simulink model "Australian14gen_forming_inertia"  (R2017b)
settings: Solver=ode23tb  StartTime=0.0  StopTime=100  FixedStep=1e-3  RelTol=1e-3  AbsTol=1e-3  EnableMultiTasking=on
PreLoadFcn:
  | dataaustralian14gen
values from neighbouring files (symbols this model uses):
  bus_v = [ 101	15 ... (first row only)    [dataaustralian14gen.m]
  c_fil = 1e-5*ones(15,1)    [dataaustralian14gen.m]
  comp = [ 1	211	0	0 ... (first row only)    [dataaustralian14gen.m]
  dist = sys.follin.dist    [main_following.m]    (also in main_forming.m = sys.formin.dist)
  Exc = [ 101	0	 200	0.1	    13.25  2.5	 0	0       0       0       0       0 ... (first row only)    [dataaustralian14gen.m]
  FH = 13    [dataaustralian14gen.m]
  FI = 1    [dataaustralian14gen.m]
  FL = .1    (= 0.1)    [dataaustralian14gen.m]
  G_data = [ 101	333.3	15	3.6	0.14	1.1	0.65	0.25	8.5     0.25	0.05	0       0       0.25	0.2 	0 ... (first row only)    [dataaustralian14gen.m]
  KH = 120    [dataaustralian14gen.m]
  KI = 10    [dataaustralian14gen.m]
  KL = 10    [dataaustralian14gen.m]
  Kvsc = 0*Kvsc    [dataaustralian14gen.m]    (also in optimgains.mat = [-4.89904313526 -21.043852985 -7.4754770322 -20.8245159401 -)
  l_fil = 5e-3*ones(15,1)    [dataaustralian14gen.m]
  line = [ 102	217	0.0084	0.0667	0.817	330	1 ... (first row only)    [dataaustralian14gen.m]
  load_mag = load_case4    [dataaustralian14gen.m]
  p = p_case4    [dataaustralian14gen.m]
  Pinit = [0.405553120017514,0.262363656270440,0.245287066765904,0.511573619715646,0.238910511748616,0.266289198874107,0.405451933295266,0.301363467877759,0.299904641553078,0.238601214125575,0.201576196829353,0.166515071179716,0.281316548159335,0.249279775700722,0.436119451429005]    [dataaustralian14gen.m]
  PSSMODEL = 1    [dataaustralian14gen.m]
  r_fil = 5e-1*ones(15,1)    [dataaustralian14gen.m]
  trans = [ 1	101	102	15	330	333.3	12	12 ... (first row only)    [dataaustralian14gen.m]
undefined symbols (not defined in the file or in its folder): D1, Delta, sys, thetavsc0
libraries: powerlib x399, Library x15, sps_avr x10, powerlib_extras x5
(part 1 of 4)
Description:
  | SimPowerSystem model of the Simplified 14-Generator model
  | of the SE Australian Power System developed by Mike Gibbard & David Vowles,
  | School of Electrical & Electronic Engineering, The university of Adelaide, south australia)
  | 
  | SimPowerSystems model and validations by Ali Moeini and Innocent Kamwa,
  | IREQ, Hydro-Québec, Canada
settings Model: Creator=IREQ  LastModifiedBy=dominic
settings DataIOCC: LimitDataPoints=on  SaveFormat=Array
settings OptimizationCC: ExpressionDepthLimit=2147483647  LifeSpan=inf
settings DebuggingCC: UnderspecifiedInitializationDetection=Classic  MergeDetectMultiDrivingBlocksExec=none  IgnoredZcDiagnostic=none  SolverPrmCheckMsg=warning  UnconnectedInputMsg=none  UnconnectedOutputMsg=none  UnconnectedLineMsg=none  StateNameClashWarn=warning  SFUnexpectedBacktrackingDiag=warning  SFNoUnconditionalDefaultTransitionDiag=warning  SFExecutionAtInitializationDiag=none
settings HardwareCC: ProdBitPerPointer=32  ProdBitPerSizeT=32  ProdBitPerPtrDiffT=32  ProdLargestAtomicFloat=None  ProdIntDivRoundTo=Undefined  ProdEndianess=Unspecified  ProdWordSize=32  ProdHWDeviceType=32-bit Generic
settings ModelReferenceCC: PropagateSignalLabelsOutOfModel=off
settings CodeAppCC: StateflowObjectComments=on
settings GRTTargetCC: TargetLangStandard=C89/C90 (ANSI)  GeneratePreprocessorConditionals=Disable all
settings ConfigComp: CovMetricSettings=dw  CovHtmlReporting=on  CovSaveCumulativeToWorkspaceVar=on  CovSaveSingleToWorkspaceVar=on  CovExternalEMLEnable=off  CovSFcnEnable=off
settings SimscapeCC: SimscapeNormalizeSystem=off

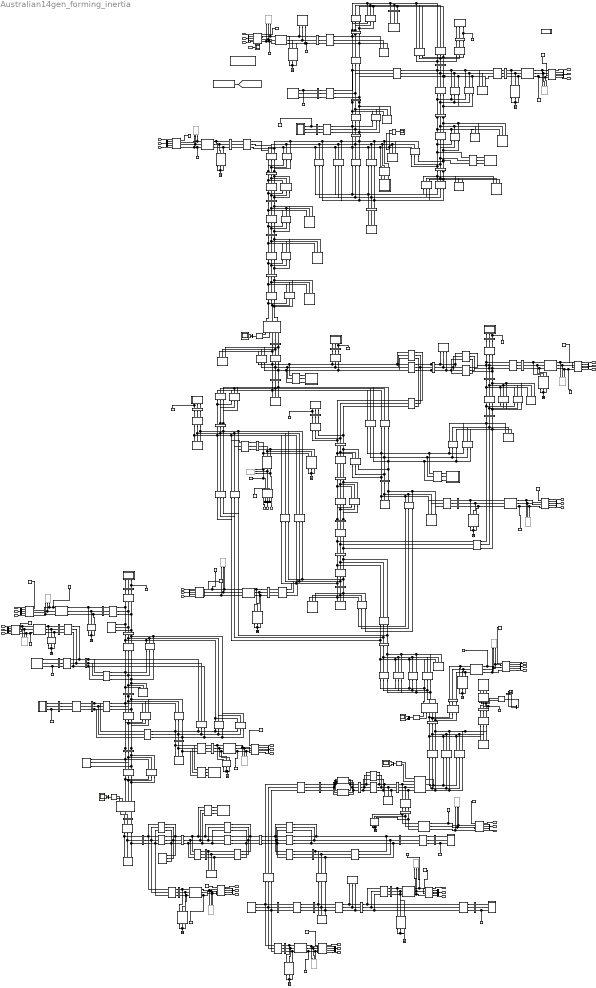
== system Australian14gen_forming_inertia ==
  1 : powerlib/Elements/Three-Phase Series RLC Branch  LConnTagsString=A|B|C  RConnTagsString=A|B|C  BranchType=C  Resistance=0  Inductance=0  Capacitance=1/(0.0337)/(2*pi*50)*(330^2/100)  Measurements=None
  15kV 1500MVA11 : powerlib/Elements/Three-Phase Series RLC Branch  LConnTagsString=A|B|C  RConnTagsString=A|B|C  BranchType=RL  Resistance=r_fil(1)  Inductance=l_fil(1)  Capacitance=[]  Measurements=None
  2 : powerlib/Elements/Three-Phase Series RLC Branch  LConnTagsString=A|B|C  RConnTagsString=A|B|C  BranchType=C  Resistance=0  Inductance=0  Capacitance=1/(0.0337)/(2*pi*50)*(330^2/100)  Measurements=None
  20kV 2000MVA : powerlib/Elements/Three-Phase Series RLC Branch  LConnTagsString=A|B|C  RConnTagsString=A|B|C  BranchType=RL  Resistance=r_fil(12)  Inductance=l_fil(12)  Capacitance=[]  Measurements=None
  20kV 2000MVA1 : powerlib/Elements/Three-Phase Series RLC Branch  LConnTagsString=A|B|C  RConnTagsString=A|B|C  BranchType=RL  Resistance=r_fil(10)  Inductance=l_fil(10)  Capacitance=[]  Measurements=None
  20kV 2000MVA10 : powerlib/Elements/Three-Phase Series RLC Branch  LConnTagsString=A|B|C  RConnTagsString=A|B|C  BranchType=RL  Resistance=r_fil(6)  Inductance=l_fil(6)  Capacitance=[]  Measurements=None
  20kV 2000MVA11 : powerlib/Elements/Three-Phase Series RLC Branch  LConnTagsString=A|B|C  RConnTagsString=A|B|C  BranchType=RL  Resistance=r_fil(14)  Inductance=l_fil(14)  Capacitance=[]  Measurements=None
  20kV 2000MVA12 : powerlib/Elements/Three-Phase Series RLC Branch  LConnTagsString=A|B|C  RConnTagsString=A|B|C  BranchType=RL  Resistance=r_fil(13)  Inductance=l_fil(13)  Capacitance=[]  Measurements=None
  20kV 2000MVA13 : powerlib/Elements/Three-Phase Series RLC Branch  LConnTagsString=A|B|C  RConnTagsString=A|B|C  BranchType=RL  Resistance=r_fil(15)  Inductance=l_fil(15)  Capacitance=[]  Measurements=None
  20kV 2000MVA14 : powerlib/Elements/Three-Phase Series RLC Branch  LConnTagsString=A|B|C  RConnTagsString=A|B|C  BranchType=C  Resistance=20^2/2000  Inductance=20^2/2000  Capacitance=c_fil(10)  Measurements=None
  20kV 2000MVA15 : powerlib/Elements/Three-Phase Series RLC Branch  LConnTagsString=A|B|C  RConnTagsString=A|B|C  BranchType=C  Resistance=20^2/2000  Inductance=20^2/2000  Capacitance=c_fil(11)  Measurements=None
  20kV 2000MVA16 : powerlib/Elements/Three-Phase Series RLC Branch  LConnTagsString=A|B|C  RConnTagsString=A|B|C  BranchType=C  Resistance=20^2/2000  Inductance=20^2/2000  Capacitance=c_fil(2)  Measurements=None
  20kV 2000MVA17 : powerlib/Elements/Three-Phase Series RLC Branch  LConnTagsString=A|B|C  RConnTagsString=A|B|C  BranchType=C  Resistance=20^2/2000  Inductance=20^2/2000  Capacitance=c_fil(3)  Measurements=None
  20kV 2000MVA18 : powerlib/Elements/Three-Phase Series RLC Branch  LConnTagsString=A|B|C  RConnTagsString=A|B|C  BranchType=C  Resistance=20^2/2000  Inductance=20^2/2000  Capacitance=c_fil(1)  Measurements=None
  20kV 2000MVA19 : powerlib/Elements/Three-Phase Series RLC Branch  LConnTagsString=A|B|C  RConnTagsString=A|B|C  BranchType=C  Resistance=20^2/2000  Inductance=20^2/2000  Capacitance=c_fil(8)  Measurements=None
  20kV 2000MVA2 : powerlib/Elements/Three-Phase Series RLC Branch  LConnTagsString=A|B|C  RConnTagsString=A|B|C  BranchType=RL  Resistance=r_fil(11)  Inductance=l_fil(11)  Capacitance=[]  Measurements=None
  20kV 2000MVA20 : powerlib/Elements/Three-Phase Series RLC Branch  LConnTagsString=A|B|C  RConnTagsString=A|B|C  BranchType=C  Resistance=20^2/2000  Inductance=20^2/2000  Capacitance=c_fil(9)  Measurements=None
  20kV 2000MVA21 : powerlib/Elements/Three-Phase Series RLC Branch  LConnTagsString=A|B|C  RConnTagsString=A|B|C  BranchType=C  Resistance=20^2/2000  Inductance=20^2/2000  Capacitance=c_fil(12)  Measurements=None
  20kV 2000MVA22 : powerlib/Elements/Three-Phase Series RLC Branch  LConnTagsString=A|B|C  RConnTagsString=A|B|C  BranchType=C  Resistance=20^2/2000  Inductance=20^2/2000  Capacitance=c_fil(5)  Measurements=None
  20kV 2000MVA23 : powerlib/Elements/Three-Phase Series RLC Branch  LConnTagsString=A|B|C  RConnTagsString=A|B|C  BranchType=C  Resistance=20^2/2000  Inductance=20^2/2000  Capacitance=c_fil(4)  Measurements=None
  20kV 2000MVA24 : powerlib/Elements/Three-Phase Series RLC Branch  LConnTagsString=A|B|C  RConnTagsString=A|B|C  BranchType=C  Resistance=20^2/2000  Inductance=20^2/2000  Capacitance=c_fil(6)  Measurements=None
  20kV 2000MVA25 : powerlib/Elements/Three-Phase Series RLC Branch  LConnTagsString=A|B|C  RConnTagsString=A|B|C  BranchType=C  Resistance=20^2/2000  Inductance=20^2/2000  Capacitance=c_fil(7)  Measurements=None
  20kV 2000MVA26 : powerlib/Elements/Three-Phase Series RLC Branch  LConnTagsString=A|B|C  RConnTagsString=A|B|C  BranchType=C  Resistance=20^2/2000  Inductance=20^2/2000  Capacitance=c_fil(15)  Measurements=None
  20kV 2000MVA27 : powerlib/Elements/Three-Phase Series RLC Branch  LConnTagsString=A|B|C  RConnTagsString=A|B|C  BranchType=C  Resistance=20^2/2000  Inductance=20^2/2000  Capacitance=c_fil(14)  Measurements=None
  20kV 2000MVA28 : powerlib/Elements/Three-Phase Series RLC Branch  LConnTagsString=A|B|C  RConnTagsString=A|B|C  BranchType=C  Resistance=20^2/2000  Inductance=20^2/2000  Capacitance=c_fil(13)  Measurements=None
  20kV 2000MVA3 : powerlib/Elements/Three-Phase Series RLC Branch  LConnTagsString=A|B|C  RConnTagsString=A|B|C  BranchType=RL  Resistance=r_fil(2)  Inductance=l_fil(2)  Capacitance=[]  Measurements=None
  20kV 2000MVA4 : powerlib/Elements/Three-Phase Series RLC Branch  LConnTagsString=A|B|C  RConnTagsString=A|B|C  BranchType=RL  Resistance=r_fil(3)  Inductance=l_fil(3)  Capacitance=[]  Measurements=None
  20kV 2000MVA5 : powerlib/Elements/Three-Phase Series RLC Branch  LConnTagsString=A|B|C  RConnTagsString=A|B|C  BranchType=RL  Resistance=r_fil(5)  Inductance=l_fil(5)  Capacitance=[]  Measurements=None
  20kV 2000MVA6 : powerlib/Elements/Three-Phase Series RLC Branch  LConnTagsString=A|B|C  RConnTagsString=A|B|C  BranchType=RL  Resistance=r_fil(4)  Inductance=l_fil(4)  Capacitance=[]  Measurements=None
  20kV 2000MVA7 : powerlib/Elements/Three-Phase Series RLC Branch  LConnTagsString=A|B|C  RConnTagsString=A|B|C  BranchType=RL  Resistance=r_fil(9)  Inductance=l_fil(9)  Capacitance=[]  Measurements=None
  20kV 2000MVA8 : powerlib/Elements/Three-Phase Series RLC Branch  LConnTagsString=A|B|C  RConnTagsString=A|B|C  BranchType=RL  Resistance=r_fil(8)  Inductance=l_fil(8)  Capacitance=[]  Measurements=None
  20kV 2000MVA9 : powerlib/Elements/Three-Phase Series RLC Branch  LConnTagsString=A|B|C  RConnTagsString=A|B|C  BranchType=RL  Resistance=r_fil(7)  Inductance=l_fil(7)  Capacitance=[]  Measurements=None
  3-Phase Active & Reactive Power (Phasor Type){1..5} (5 alike) : powerlib_extras/Phasor Library/3-Phase Active & Reactive Power (Phasor Type)
  3-Phase Dynamic Load3 : powerlib/Elements/Three-Phase Dynamic Load  NominalVoltage=[ 15e3 50 ]  ActiveReactivePowers=[-5.4e+08 -4.56e+06]  PositiveSequence=[0.999196 -2.87767]  ExternalControl=off  NpNq="[0  0]"  TimeConstants=[0 0 0 0]  MinimumVoltage=0.01  Tfilter=1e-2  LoadFlowParameters=[4 50000000 0 0 25000000]
      settings: SourceProductName=Simscape Power Systems  SourceProductBaseCode=PS
  3-Phase Dynamic Load4 : powerlib/Elements/Three-Phase Dynamic Load  NominalVoltage=[ 15e3 50 ]  ActiveReactivePowers=[-1000 -8.47033e-14]  PositiveSequence=[1.08335 6.60259]  ExternalControl=off  NpNq="[0  0]"  TimeConstants=[0 0 0 0]  MinimumVoltage=0.01  Tfilter=1e-2  LoadFlowParameters=[4 50000000 0 0 25000000]
      settings: SourceProductName=Simscape Power Systems  SourceProductBaseCode=PS
  B101 : powerlib/Measurements/Three-Phase V-I Measurement  VoltageMeasurement=phase-to-ground  SetLabelV=on  LabelV=Vabc_B101  Vpu=off  VpuLL=off  CurrentMeasurement=no  SetLabelI=on  LabelI=Iabc_B101  Ipu=off  Pbase=100e6  Vbase=bus_v(1,2)*e3  OutputType=Magnitude  PhasorSimulation=on  PSBequivalent=0
  B102 : powerlib/Measurements/Three-Phase V-I Measurement  VoltageMeasurement=phase-to-ground  SetLabelV=on  LabelV=Vabc_B102  Vpu=off  VpuLL=off  CurrentMeasurement=yes  SetLabelI=on  LabelI=Iabc_B102  Ipu=off  Pbase=100e6  Vbase=bus_v(2,2)*e3  OutputType=Complex  PhasorSimulation=on  PSBequivalent=0
  B102_vi : powerlib/Measurements/Three-Phase V-I Measurement  VoltageMeasurement=phase-to-phase  SetLabelV=on  LabelV=Vabc_B102_vi  Vpu=off  VpuLL=off  CurrentMeasurement=no  SetLabelI=on  LabelI=Iabc_B101  Ipu=off  Pbase=100e6  Vbase=bus_v(1,2)*e3  OutputType=Complex  PhasorSimulation=on  PSBequivalent=0
  B201 : powerlib/Measurements/Three-Phase V-I Measurement  VoltageMeasurement=phase-to-phase  SetLabelV=on  LabelV=Vabc_B201  Vpu=off  VpuLL=off  CurrentMeasurement=no  SetLabelI=on  LabelI=Iabc_B201  Ipu=off  Pbase=100e6  Vbase=bus_v(3,2)*e3  OutputType=Complex  PhasorSimulation=on  PSBequivalent=0
  B202 : powerlib/Measurements/Three-Phase V-I Measurement  VoltageMeasurement=phase-to-phase  SetLabelV=on  LabelV=Vabc_B202  Vpu=off  VpuLL=off  CurrentMeasurement=no  SetLabelI=on  LabelI=Iabc_B202  Ipu=off  Pbase=100e6  Vbase=bus_v(4,2)*e3  OutputType=Complex  PhasorSimulation=on  PSBequivalent=0
  B203 : powerlib/Measurements/Three-Phase V-I Measurement  VoltageMeasurement=phase-to-phase  SetLabelV=on  LabelV=Vabc_B203  Vpu=off  VpuLL=off  CurrentMeasurement=no  SetLabelI=on  LabelI=Iabc_B203  Ipu=off  Pbase=100e6  Vbase=bus_v(5,2)*e3  OutputType=Complex  PhasorSimulation=on  PSBequivalent=0
  B204 : powerlib/Measurements/Three-Phase V-I Measurement  VoltageMeasurement=phase-to-phase  SetLabelV=on  LabelV=Vabc_B204  Vpu=off  VpuLL=off  CurrentMeasurement=no  SetLabelI=on  LabelI=Iabc_B204  Ipu=off  Pbase=100e6  Vbase=bus_v(6,2)*e3  OutputType=Complex  PhasorSimulation=on  PSBequivalent=0
  B205 : powerlib/Measurements/Three-Phase V-I Measurement  VoltageMeasurement=phase-to-ground  SetLabelV=on  LabelV=Vabc_B205  Vpu=off  VpuLL=off  CurrentMeasurement=yes  SetLabelI=on  LabelI=Iabc_B205  Ipu=off  Pbase=100e6  Vbase=bus_v(7,2)*e3  OutputType=Complex  PhasorSimulation=on  PSBequivalent=0
  B206 : powerlib/Measurements/Three-Phase V-I Measurement  VoltageMeasurement=phase-to-ground  SetLabelV=on  LabelV=Vabc_B206  Vpu=off  VpuLL=off  CurrentMeasurement=yes  SetLabelI=on  LabelI=Iabc_B206  Ipu=off  Pbase=100e6  Vbase=bus_v(8,2)*e3  OutputType=Complex  PhasorSimulation=on  PSBequivalent=0
  B207 : powerlib/Measurements/Three-Phase V-I Measurement  VoltageMeasurement=phase-to-ground  SetLabelV=on  LabelV=Vabc_B207  Vpu=off  VpuLL=off  CurrentMeasurement=yes  SetLabelI=on  LabelI=Iabc_B207  Ipu=off  Pbase=100e6  Vbase=138e3  OutputType=Complex  PhasorSimulation=on  PSBequivalent=0
  B208 : powerlib/Measurements/Three-Phase V-I Measurement  VoltageMeasurement=phase-to-ground  SetLabelV=on  LabelV=Vabc_B208  Vpu=off  VpuLL=off  CurrentMeasurement=yes  SetLabelI=on  LabelI=Iabc_B208  Ipu=off  Pbase=100e6  Vbase=138e3  OutputType=Complex  PhasorSimulation=on  PSBequivalent=0
  B208_vi : powerlib/Measurements/Three-Phase V-I Measurement  VoltageMeasurement=phase-to-phase  SetLabelV=on  LabelV=Vabc_B208_vi  Vpu=off  VpuLL=off  CurrentMeasurement=no  SetLabelI=on  LabelI=Iabc_B203  Ipu=off  Pbase=100e6  Vbase=bus_v(5,2)*e3  OutputType=Complex  PhasorSimulation=on  PSBequivalent=0
  B209 : powerlib/Measurements/Three-Phase V-I Measurement  VoltageMeasurement=phase-to-ground  SetLabelV=on  LabelV=Vabc_B209  Vpu=off  VpuLL=off  CurrentMeasurement=yes  SetLabelI=on  LabelI=Iabc_B209  Ipu=off  Pbase=100e6  Vbase=138e3  OutputType=Complex  PhasorSimulation=on  PSBequivalent=0
  B210 : powerlib/Measurements/Three-Phase V-I Measurement  VoltageMeasurement=phase-to-ground  SetLabelV=on  LabelV=Vabc_B210  Vpu=off  VpuLL=off  CurrentMeasurement=yes  SetLabelI=on  LabelI=Iabc_B210  Ipu=off  Pbase=100e6  Vbase=138e3  OutputType=Complex  PhasorSimulation=on  PSBequivalent=0
  B211 : powerlib/Measurements/Three-Phase V-I Measurement  VoltageMeasurement=phase-to-ground  SetLabelV=on  LabelV=Vabc_B211  Vpu=off  VpuLL=off  CurrentMeasurement=yes  SetLabelI=on  LabelI=Iabc_B211  Ipu=off  Pbase=100e6  Vbase=138e3  OutputType=Complex  PhasorSimulation=on  PSBequivalent=0
  B212 : powerlib/Measurements/Three-Phase V-I Measurement  VoltageMeasurement=phase-to-ground  SetLabelV=on  LabelV=Vabc_B212  Vpu=off  VpuLL=off  CurrentMeasurement=yes  SetLabelI=on  LabelI=Iabc_B212  Ipu=off  Pbase=100e6  Vbase=138e3  OutputType=Complex  PhasorSimulation=on  PSBequivalent=0
  B212_vi : powerlib/Measurements/Three-Phase V-I Measurement  VoltageMeasurement=phase-to-phase  SetLabelV=on  LabelV=Vabc_B212_vi  Vpu=off  VpuLL=off  CurrentMeasurement=no  SetLabelI=on  LabelI=Iabc_B203  Ipu=off  Pbase=100e6  Vbase=bus_v(5,2)*e3  OutputType=Complex  PhasorSimulation=on  PSBequivalent=0
  B213 : powerlib/Measurements/Three-Phase V-I Measurement  VoltageMeasurement=phase-to-ground  SetLabelV=on  LabelV=Vabc_B213  Vpu=off  VpuLL=off  CurrentMeasurement=yes  SetLabelI=on  LabelI=Iabc_B213  Ipu=off  Pbase=100e6  Vbase=138e3  OutputType=Complex  PhasorSimulation=on  PSBequivalent=0
  B214 : powerlib/Measurements/Three-Phase V-I Measurement  VoltageMeasurement=phase-to-ground  SetLabelV=on  LabelV=Vabc_B214  Vpu=off  VpuLL=off  CurrentMeasurement=yes  SetLabelI=on  LabelI=Iabc_B214  Ipu=off  Pbase=100e6  Vbase=138e3  OutputType=Complex  PhasorSimulation=on  PSBequivalent=0
  B215 : powerlib/Measurements/Three-Phase V-I Measurement  VoltageMeasurement=phase-to-ground  SetLabelV=on  LabelV=Vabc_B215  Vpu=off  VpuLL=off  CurrentMeasurement=yes  SetLabelI=on  LabelI=Iabc_B215  Ipu=off  Pbase=100e6  Vbase=138e3  OutputType=Complex  PhasorSimulation=on  PSBequivalent=0
  B215_vi : powerlib/Measurements/Three-Phase V-I Measurement  VoltageMeasurement=phase-to-phase  SetLabelV=on  LabelV=Vabc_B215_vi  Vpu=off  VpuLL=off  CurrentMeasurement=no  SetLabelI=on  LabelI=Iabc_B215  Ipu=off  Pbase=100e6  Vbase=138e3  OutputType=Complex  PhasorSimulation=on  PSBequivalent=0
  B216 : powerlib/Measurements/Three-Phase V-I Measurement  VoltageMeasurement=phase-to-ground  SetLabelV=on  LabelV=Vabc_B216  Vpu=off  VpuLL=off  CurrentMeasurement=yes  SetLabelI=on  LabelI=Iabc_B216  Ipu=off  Pbase=100e6  Vbase=138e3  OutputType=Complex  PhasorSimulation=on  PSBequivalent=0
  B216_vi : powerlib/Measurements/Three-Phase V-I Measurement  VoltageMeasurement=phase-to-phase  SetLabelV=on  LabelV=Vabc_B216_vi  Vpu=off  VpuLL=off  CurrentMeasurement=no  SetLabelI=off  LabelI=Iabc_B216  Ipu=off  Pbase=100e6  Vbase=138e3  OutputType=Complex  PhasorSimulation=on  PSBequivalent=0
  B217 : powerlib/Measurements/Three-Phase V-I Measurement  VoltageMeasurement=phase-to-ground  SetLabelV=on  LabelV=Vabc_B217  Vpu=off  VpuLL=off  CurrentMeasurement=yes  SetLabelI=on  LabelI=Iabc_B217  Ipu=off  Pbase=100e6  Vbase=138e3  OutputType=Complex  PhasorSimulation=on  PSBequivalent=0
  B301 : powerlib/Measurements/Three-Phase V-I Measurement  VoltageMeasurement=phase-to-phase  SetLabelV=on  LabelV=Vabc_B301  Vpu=off  VpuLL=off  CurrentMeasurement=no  SetLabelI=on  LabelI=Iabc_B301  Ipu=off  Pbase=100e6  Vbase=138e3  OutputType=Complex  PhasorSimulation=on  PSBequivalent=0
  B302 : powerlib/Measurements/Three-Phase V-I Measurement  VoltageMeasurement=phase-to-phase  SetLabelV=on  LabelV=Vabc_B302  Vpu=off  VpuLL=off  CurrentMeasurement=no  SetLabelI=on  LabelI=Iabc_B302  Ipu=off  Pbase=100e6  Vbase=138e3  OutputType=Complex  PhasorSimulation=on  PSBequivalent=0
  B303 : powerlib/Measurements/Three-Phase V-I Measurement  VoltageMeasurement=phase-to-ground  SetLabelV=on  LabelV=Vabc_B303  Vpu=off  VpuLL=off  CurrentMeasurement=yes  SetLabelI=on  LabelI=Iabc_B303  Ipu=off  Pbase=100e6  Vbase=138e3  OutputType=Complex  PhasorSimulation=on  PSBequivalent=0
  B304 : powerlib/Measurements/Three-Phase V-I Measurement  VoltageMeasurement=phase-to-ground  SetLabelV=on  LabelV=Vabc_B304  Vpu=off  VpuLL=off  CurrentMeasurement=yes  SetLabelI=on  LabelI=Iabc_B304  Ipu=off  Pbase=100e6  Vbase=138e3  OutputType=Complex  PhasorSimulation=on  PSBequivalent=0
  B305 : powerlib/Measurements/Three-Phase V-I Measurement  VoltageMeasurement=phase-to-ground  SetLabelV=on  LabelV=Vabc_B305  Vpu=off  VpuLL=off  CurrentMeasurement=yes  SetLabelI=on  LabelI=Iabc_B305  Ipu=off  Pbase=100e6  Vbase=138e3  OutputType=Complex  PhasorSimulation=on  PSBequivalent=0
  B306 : powerlib/Measurements/Three-Phase V-I Measurement  VoltageMeasurement=phase-to-ground  SetLabelV=on  LabelV=Vabc_B306  Vpu=off  VpuLL=off  CurrentMeasurement=yes  SetLabelI=on  LabelI=Iabc_B306  Ipu=off  Pbase=100e6  Vbase=138e3  OutputType=Complex  PhasorSimulation=on  PSBequivalent=0
  B307 : powerlib/Measurements/Three-Phase V-I Measurement  VoltageMeasurement=phase-to-ground  SetLabelV=on  LabelV=Vabc_B307  Vpu=off  VpuLL=off  CurrentMeasurement=yes  SetLabelI=on  LabelI=Iabc_B307  Ipu=off  Pbase=100e6  Vbase=138e3  OutputType=Complex  PhasorSimulation=on  PSBequivalent=0
  B308 : powerlib/Measurements/Three-Phase V-I Measurement  VoltageMeasurement=phase-to-ground  SetLabelV=on  LabelV=Vabc_B308  Vpu=off  VpuLL=off  CurrentMeasurement=yes  SetLabelI=on  LabelI=Iabc_B308  Ipu=off  Pbase=100e6  Vbase=138e3  OutputType=Complex  PhasorSimulation=on  PSBequivalent=0
  B308_vi : powerlib/Measurements/Three-Phase V-I Measurement  VoltageMeasurement=phase-to-phase  SetLabelV=on  LabelV=Vabc_B308_vi  Vpu=off  VpuLL=off  CurrentMeasurement=no  SetLabelI=on  LabelI=Iabc_B301  Ipu=off  Pbase=100e6  Vbase=138e3  OutputType=Complex  PhasorSimulation=on  PSBequivalent=0
  B309 : powerlib/Measurements/Three-Phase V-I Measurement  VoltageMeasurement=phase-to-ground  SetLabelV=on  LabelV=Vabc_B309  Vpu=off  VpuLL=off  CurrentMeasurement=yes  SetLabelI=on  LabelI=Iabc_B309  Ipu=off  Pbase=100e6  Vbase=138e3  OutputType=Complex  PhasorSimulation=on  PSBequivalent=0
  B309_vi : powerlib/Measurements/Three-Phase V-I Measurement  VoltageMeasurement=phase-to-phase  SetLabelV=on  LabelV=Vabc_B309_vi  Vpu=off  VpuLL=off  CurrentMeasurement=no  SetLabelI=off  LabelI=Iabc_B309  Ipu=off  Pbase=100e6  Vbase=138e3  OutputType=Complex  PhasorSimulation=on  PSBequivalent=0
  B310 : powerlib/Measurements/Three-Phase V-I Measurement  VoltageMeasurement=phase-to-ground  SetLabelV=on  LabelV=Vabc_B310  Vpu=off  VpuLL=off  CurrentMeasurement=yes  SetLabelI=on  LabelI=Iabc_B310  Ipu=off  Pbase=100e6  Vbase=138e3  OutputType=Complex  PhasorSimulation=on  PSBequivalent=0
  B311 : powerlib/Measurements/Three-Phase V-I Measurement  VoltageMeasurement=phase-to-ground  SetLabelV=on  LabelV=Vabc_B311  Vpu=off  VpuLL=off  CurrentMeasurement=yes  SetLabelI=on  LabelI=Iabc_B311  Ipu=off  Pbase=100e6  Vbase=138e3  OutputType=Complex  PhasorSimulation=on  PSBequivalent=0
  B312 : powerlib/Measurements/Three-Phase V-I Measurement  VoltageMeasurement=phase-to-ground  SetLabelV=on  LabelV=Vabc_B312  Vpu=off  VpuLL=off  CurrentMeasurement=yes  SetLabelI=on  LabelI=Iabc_B312  Ipu=off  Pbase=100e6  Vbase=138e3  OutputType=Complex  PhasorSimulation=on  PSBequivalent=0
  B312_vi : powerlib/Measurements/Three-Phase V-I Measurement  VoltageMeasurement=phase-to-phase  SetLabelV=on  LabelV=Vabc_B312_vi  Vpu=off  VpuLL=off  CurrentMeasurement=no  SetLabelI=off  LabelI=Iabc_B312_vi  Ipu=off  Pbase=100e6  Vbase=138e3  OutputType=Complex  PhasorSimulation=on  PSBequivalent=0
  B313 : powerlib/Measurements/Three-Phase V-I Measurement  VoltageMeasurement=phase-to-ground  SetLabelV=on  LabelV=Vabc_B313  Vpu=off  VpuLL=off  CurrentMeasurement=yes  SetLabelI=on  LabelI=Iabc_B313  Ipu=off  Pbase=100e6  Vbase=138e3  OutputType=Complex  PhasorSimulation=on  PSBequivalent=0
  B314 : powerlib/Measurements/Three-Phase V-I Measurement  VoltageMeasurement=phase-to-ground  SetLabelV=on  LabelV=Vabc_B314  Vpu=off  VpuLL=off  CurrentMeasurement=yes  SetLabelI=on  LabelI=Iabc_B314  Ipu=off  Pbase=100e6  Vbase=138e3  OutputType=Complex  PhasorSimulation=on  PSBequivalent=0
  B314_vi : powerlib/Measurements/Three-Phase V-I Measurement  VoltageMeasurement=phase-to-phase  SetLabelV=on  LabelV=Vabc_B314_vi  Vpu=off  VpuLL=off  CurrentMeasurement=no  SetLabelI=off  LabelI=Iabc_B314_vi  Ipu=off  Pbase=100e6  Vbase=138e3  OutputType=Complex  PhasorSimulation=on  PSBequivalent=0
  B315 : powerlib/Measurements/Three-Phase V-I Measurement  VoltageMeasurement=phase-to-ground  SetLabelV=on  LabelV=Vabc_B315  Vpu=off  VpuLL=off  CurrentMeasurement=yes  SetLabelI=on  LabelI=Iabc_B315  Ipu=off  Pbase=100e6  Vbase=138e3  OutputType=Complex  PhasorSimulation=on  PSBequivalent=0
  B401 : powerlib/Measurements/Three-Phase V-I Measurement  VoltageMeasurement=phase-to-phase  SetLabelV=on  LabelV=Vabc_B401  Vpu=off  VpuLL=off  CurrentMeasurement=no  SetLabelI=on  LabelI=Iabc_B401  Ipu=off  Pbase=100e6  Vbase=138e3  OutputType=Complex  PhasorSimulation=on  PSBequivalent=0
  B402 : powerlib/Measurements/Three-Phase V-I Measurement  VoltageMeasurement=phase-to-ground  SetLabelV=on  LabelV=Vabc_B402  Vpu=off  VpuLL=off  CurrentMeasurement=no  SetLabelI=off  LabelI=Iabc_B402  Ipu=off  Pbase=100e6  Vbase=138e3  OutputType=Magnitude  PhasorSimulation=on  PSBequivalent=0
  B403_vi : powerlib/Measurements/Three-Phase V-I Measurement  VoltageMeasurement=phase-to-phase  SetLabelV=on  LabelV=Vabc_B403_vi  Vpu=off  VpuLL=off  CurrentMeasurement=no  SetLabelI=on  LabelI=Iabc_B403  Ipu=off  Pbase=100e6  Vbase=138e3  OutputType=Complex  PhasorSimulation=on  PSBequivalent=0
  B404 : powerlib/Measurements/Three-Phase V-I Measurement  VoltageMeasurement=phase-to-phase  SetLabelV=on  LabelV=Vabc_B404  Vpu=off  VpuLL=off  CurrentMeasurement=no  SetLabelI=on  LabelI=Iabc_B404  Ipu=off  Pbase=100e6  Vbase=138e3  OutputType=Complex  PhasorSimulation=on  PSBequivalent=0
  B405 : powerlib/Measurements/Three-Phase V-I Measurement  VoltageMeasurement=phase-to-ground  SetLabelV=on  LabelV=Vabc_B405  Vpu=off  VpuLL=off  CurrentMeasurement=yes  SetLabelI=on  LabelI=Iabc_B405  Ipu=off  Pbase=100e6  Vbase=138e3  OutputType=Complex  PhasorSimulation=on  PSBequivalent=0
  B405_vi : powerlib/Measurements/Three-Phase V-I Measurement  VoltageMeasurement=phase-to-phase  SetLabelV=on  LabelV=Vabc_B405_vi  Vpu=off  VpuLL=off  CurrentMeasurement=no  SetLabelI=on  LabelI=Iabc_B404  Ipu=off  Pbase=100e6  Vbase=138e3  OutputType=Complex  PhasorSimulation=on  PSBequivalent=0
  B406 : powerlib/Measurements/Three-Phase V-I Measurement  VoltageMeasurement=phase-to-ground  SetLabelV=on  LabelV=Vabc_B406  Vpu=off  VpuLL=off  CurrentMeasurement=yes  SetLabelI=on  LabelI=Iabc_B406  Ipu=off  Pbase=100e6  Vbase=138e3  OutputType=Complex  PhasorSimulation=on  PSBequivalent=0
  B407 : powerlib/Measurements/Three-Phase V-I Measurement  VoltageMeasurement=phase-to-ground  SetLabelV=on  LabelV=Vabc_B407  Vpu=off  VpuLL=off  CurrentMeasurement=yes  SetLabelI=on  LabelI=Iabc_B407  Ipu=off  Pbase=100e6  Vbase=138e3  OutputType=Complex  PhasorSimulation=on  PSBequivalent=0
  B408 : powerlib/Measurements/Three-Phase V-I Measurement  VoltageMeasurement=phase-to-ground  SetLabelV=on  LabelV=Vabc_B408  Vpu=off  VpuLL=off  CurrentMeasurement=yes  SetLabelI=on  LabelI=Iabc_B408  Ipu=off  Pbase=100e6  Vbase=138e3  OutputType=Complex  PhasorSimulation=on  PSBequivalent=0
  B409 : powerlib/Measurements/Three-Phase V-I Measurement  VoltageMeasurement=phase-to-ground  SetLabelV=on  LabelV=Vabc_B409  Vpu=off  VpuLL=off  CurrentMeasurement=yes  SetLabelI=on  LabelI=Iabc_B409  Ipu=off  Pbase=100e6  Vbase=138e3  OutputType=Complex  PhasorSimulation=on  PSBequivalent=0
  B410 : powerlib/Measurements/Three-Phase V-I Measurement  VoltageMeasurement=phase-to-ground  SetLabelV=on  LabelV=Vabc_B410  Vpu=off  VpuLL=off  CurrentMeasurement=no  SetLabelI=on  LabelI=Iabc_B410  Ipu=off  Pbase=100e6  Vbase=138e3  OutputType=Magnitude  PhasorSimulation=on  PSBequivalent=0
  B410_vi : powerlib/Measurements/Three-Phase V-I Measurement  VoltageMeasurement=phase-to-phase  SetLabelV=on  LabelV=Vabc_B410_vi  Vpu=off  VpuLL=off  CurrentMeasurement=no  SetLabelI=on  LabelI=Iabc_B401  Ipu=off  Pbase=100e6  Vbase=138e3  OutputType=Complex  PhasorSimulation=on  PSBequivalent=0
  B411 : powerlib/Measurements/Three-Phase V-I Measurement  VoltageMeasurement=phase-to-ground  SetLabelV=on  LabelV=Vabc_B411  Vpu=off  VpuLL=off  CurrentMeasurement=yes  SetLabelI=on  LabelI=Iabc_B411  Ipu=off  Pbase=100e6  Vbase=138e3  OutputType=Complex  PhasorSimulation=on  PSBequivalent=0
  B412 : powerlib/Measurements/Three-Phase V-I Measurement  VoltageMeasurement=phase-to-ground  SetLabelV=on  LabelV=Vabc_B412  Vpu=off  VpuLL=off  CurrentMeasurement=yes  SetLabelI=on  LabelI=Iabc_B412  Ipu=off  Pbase=100e6  Vbase=138e3  OutputType=Complex  PhasorSimulation=on  PSBequivalent=0
  B413 : powerlib/Measurements/Three-Phase V-I Measurement  VoltageMeasurement=phase-to-ground  SetLabelV=on  LabelV=Vabc_B413  Vpu=off  VpuLL=off  CurrentMeasurement=yes  SetLabelI=on  LabelI=Iabc_B413  Ipu=off  Pbase=100e6  Vbase=138e3  OutputType=Complex  PhasorSimulation=on  PSBequivalent=0
  B414 : powerlib/Measurements/Three-Phase V-I Measurement  VoltageMeasurement=phase-to-ground  SetLabelV=on  LabelV=Vabc_B414  Vpu=off  VpuLL=off  CurrentMeasurement=yes  SetLabelI=on  LabelI=Iabc_B414  Ipu=off  Pbase=100e6  Vbase=138e3  OutputType=Complex  PhasorSimulation=on  PSBequivalent=0
  B415 : powerlib/Measurements/Three-Phase V-I Measurement  VoltageMeasurement=phase-to-ground  SetLabelV=on  LabelV=Vabc_B415  Vpu=off  VpuLL=off  CurrentMeasurement=yes  SetLabelI=on  LabelI=Iabc_B415  Ipu=off  Pbase=100e6  Vbase=138e3  OutputType=Complex  PhasorSimulation=on  PSBequivalent=0
  B416 : powerlib/Measurements/Three-Phase V-I Measurement  VoltageMeasurement=phase-to-ground  SetLabelV=on  LabelV=Vabc_B416  Vpu=off  VpuLL=off  CurrentMeasurement=yes  SetLabelI=on  LabelI=Iabc_B416  Ipu=off  Pbase=100e6  Vbase=138e3  OutputType=Complex  PhasorSimulation=on  PSBequivalent=0
  B501 : powerlib/Measurements/Three-Phase V-I Measurement  VoltageMeasurement=phase-to-phase  SetLabelV=on  LabelV=Vabc_B501  Vpu=off  VpuLL=off  CurrentMeasurement=no  SetLabelI=on  LabelI=Iabc_B501  Ipu=off  Pbase=100e6  Vbase=138e3  OutputType=Complex  PhasorSimulation=on  PSBequivalent=0
  B502 : powerlib/Measurements/Three-Phase V-I Measurement  VoltageMeasurement=no  SetLabelV=on  LabelV=Vabc_B502  Vpu=off  VpuLL=off  CurrentMeasurement=no  SetLabelI=on  LabelI=Iabc_B502  Ipu=off  Pbase=100e6  Vbase=138e3  OutputType=Complex  PhasorSimulation=on  PSBequivalent=0
  B502_vi : powerlib/Measurements/Three-Phase V-I Measurement  VoltageMeasurement=phase-to-phase  SetLabelV=on  LabelV=Vabc_B502_vi  Vpu=off  VpuLL=off  CurrentMeasurement=no  SetLabelI=on  LabelI=Iabc_B502  Ipu=off  Pbase=100e6  Vbase=138e3  OutputType=Complex  PhasorSimulation=on  PSBequivalent=0
  B503 : powerlib/Measurements/Three-Phase V-I Measurement  VoltageMeasurement=phase-to-phase  SetLabelV=on  LabelV=Vabc_B503  Vpu=off  VpuLL=off  CurrentMeasurement=yes  SetLabelI=on  LabelI=Iabc_B503  Ipu=off  Pbase=100e6  Vbase=138e3  OutputType=Complex  PhasorSimulation=on  PSBequivalent=0
  B504 : powerlib/Measurements/Three-Phase V-I Measurement  VoltageMeasurement=phase-to-ground  SetLabelV=on  LabelV=Vabc_B504  Vpu=off  VpuLL=off  CurrentMeasurement=yes  SetLabelI=on  LabelI=Iabc_B504  Ipu=off  Pbase=100e6  Vbase=138e3  OutputType=Complex  PhasorSimulation=on  PSBequivalent=0
  B504_vi : powerlib/Measurements/Three-Phase V-I Measurement  VoltageMeasurement=phase-to-phase  SetLabelV=on  LabelV=Vabc_B504_vi  Vpu=off  VpuLL=off  CurrentMeasurement=no  SetLabelI=on  LabelI=Iabc_B502  Ipu=off  Pbase=100e6  Vbase=138e3  OutputType=Complex  PhasorSimulation=on  PSBequivalent=0
  B505 : powerlib/Measurements/Three-Phase V-I Measurement  VoltageMeasurement=phase-to-ground  SetLabelV=on  LabelV=Vabc_B505  Vpu=off  VpuLL=off  CurrentMeasurement=yes  SetLabelI=on  LabelI=Iabc_B505  Ipu=off  Pbase=100e6  Vbase=138e3  OutputType=Complex  PhasorSimulation=on  PSBequivalent=0
  B506 : powerlib/Measurements/Three-Phase V-I Measurement  VoltageMeasurement=phase-to-ground  SetLabelV=on  LabelV=Vabc_B506  Vpu=off  VpuLL=off  CurrentMeasurement=yes  SetLabelI=on  LabelI=Iabc_B506  Ipu=off  Pbase=100e6  Vbase=138e3  OutputType=Complex  PhasorSimulation=on  PSBequivalent=0
  B507 : powerlib/Measurements/Three-Phase V-I Measurement  VoltageMeasurement=phase-to-ground  SetLabelV=on  LabelV=Vabc_B507  Vpu=off  VpuLL=off  CurrentMeasurement=yes  SetLabelI=on  LabelI=Iabc_B507  Ipu=off  Pbase=100e6  Vbase=138e3  OutputType=Complex  PhasorSimulation=on  PSBequivalent=0
  B508 : powerlib/Measurements/Three-Phase V-I Measurement  VoltageMeasurement=phase-to-ground  SetLabelV=on  LabelV=Vabc_B508  Vpu=off  VpuLL=off  CurrentMeasurement=yes  SetLabelI=on  LabelI=Iabc_B508  Ipu=off  Pbase=100e6  Vbase=138e3  OutputType=Complex  PhasorSimulation=on  PSBequivalent=0
  B508_vi : powerlib/Measurements/Three-Phase V-I Measurement  VoltageMeasurement=phase-to-phase  SetLabelV=on  LabelV=Vabc_B508_vi  Vpu=off  VpuLL=off  CurrentMeasurement=no  SetLabelI=off  LabelI=Iabc_B503  Ipu=off  Pbase=100e6  Vbase=138e3  OutputType=Complex  PhasorSimulation=on  PSBequivalent=0
  B509 : powerlib/Measurements/Three-Phase V-I Measurement  VoltageMeasurement=phase-to-ground  SetLabelV=on  LabelV=Vabc_B3509  Vpu=off  VpuLL=off  CurrentMeasurement=yes  SetLabelI=on  LabelI=Iabc_B509  Ipu=off  Pbase=100e6  Vbase=138e3  OutputType=Complex  PhasorSimulation=on  PSBequivalent=0
  CPS402 : powerlib/Elements/Three-Phase Dynamic Load  NominalVoltage=[ 20e3 50 ]  ActiveReactivePowers=[-5.8e+08 1.015e+07]  PositiveSequence=[0.996609 23.9171]  ExternalControl=off  NpNq="[0  0]"  TimeConstants=[0 0 0 0]  MinimumVoltage=0.01  Tfilter=1e-2  LoadFlowParameters=[4 50000000 0 0 25000000]
      settings: SourceProductName=Simscape Power Systems  SourceProductBaseCode=PS
  CPS403 : powerlib/Elements/Three-Phase Dynamic Load  NominalVoltage=[ 20e3 50 ]  ActiveReactivePowers=[-9.6e+08 -3.808e+07]  PositiveSequence=[0.997203 23.5817]  ExternalControl=off  NpNq="[0  0]"  TimeConstants=[0 0 0 0]  MinimumVoltage=0.01  Tfilter=1e-2  LoadFlowParameters=[4 50000000 0 0 25000000]
      settings: SourceProductName=Simscape Power Systems  SourceProductBaseCode=PS
  Comp2-212 : powerlib/Elements/Three-Phase Parallel RLC Load  LConnTagsString=A|B|C  Configuration=Y (grounded)  NominalVoltage=(330000)*1  Vabc=[1e3 1e3 1e3]  Vabcp=[1e3 1e3 1e3]  NominalFrequency=50  UnbalancedPower=off  ActivePower=0  InductivePower=comp(2,3)*1e6  CapacitivePower=comp(2,4)*1e6  Pabc=[10e3 9e3 11e3]  QLabc=[100 90 110]  QCabc=[100 90 110]  Pabcp=[10e3 9e3 11e3]  QLabcp=[100 90 110]  QCabcp=[100 90 110]  Measurements=None  LoadType=constant Z
  Comp3-216 : powerlib/Elements/Three-Phase Parallel RLC Load  LConnTagsString=A|B|C  Configuration=Y (grounded)  NominalVoltage=(330000)*1  Vabc=[1e3 1e3 1e3]  Vabcp=[1e3 1e3 1e3]  NominalFrequency=50  UnbalancedPower=off  ActivePower=0  InductivePower=comp(3,3)*1e6  CapacitivePower=comp(3,4)*1e6  Pabc=[10e3 9e3 11e3]  QLabc=[100 90 110]  QCabc=[100 90 110]  Pabcp=[10e3 9e3 11e3]  QLabcp=[100 90 110]  QCabcp=[100 90 110]  Measurements=None  LoadType=constant Z
  Comp4-409 : powerlib/Elements/Three-Phase Parallel RLC Load  LConnTagsString=A|B|C  Configuration=Y (grounded)  NominalVoltage=(275000)*1  Vabc=[1e3 1e3 1e3]  Vabcp=[1e3 1e3 1e3]  NominalFrequency=50  UnbalancedPower=off  ActivePower=0  InductivePower=comp(4,3)*1e6  CapacitivePower=comp(4,4)*1e6  Pabc=[10e3 9e3 11e3]  QLabc=[100 90 110]  QCabc=[100 90 110]  Pabcp=[10e3 9e3 11e3]  QLabcp=[100 90 110]  QCabcp=[100 90 110]  Measurements=None  LoadType=constant Z
  Comp5-411 : powerlib/Elements/Three-Phase Parallel RLC Load  LConnTagsString=A|B|C  Configuration=Y (grounded)  NominalVoltage=(275000)*1  Vabc=[1e3 1e3 1e3]  Vabcp=[1e3 1e3 1e3]  NominalFrequency=50  UnbalancedPower=off  ActivePower=0  InductivePower=comp(5,3)*1e6  CapacitivePower=comp(5,4)*1e6  Pabc=[10e3 9e3 11e3]  QLabc=[100 90 110]  QCabc=[100 90 110]  Pabcp=[10e3 9e3 11e3]  QLabcp=[100 90 110]  QCabcp=[100 90 110]  Measurements=None  LoadType=constant Z
  Comp6-414 : powerlib/Elements/Three-Phase Parallel RLC Load  LConnTagsString=A|B|C  Configuration=Y (grounded)  NominalVoltage=(330000)*1  Vabc=[1e3 1e3 1e3]  Vabcp=[1e3 1e3 1e3]  NominalFrequency=50  UnbalancedPower=off  ActivePower=0  InductivePower=comp(6,3)*1e6  CapacitivePower=comp(6,4)*1e6  Pabc=[10e3 9e3 11e3]  QLabc=[100 90 110]  QCabc=[100 90 110]  Pabcp=[10e3 9e3 11e3]  QLabcp=[100 90 110]  QCabcp=[100 90 110]  Measurements=None  LoadType=constant Z
  Comp7-415 : powerlib/Elements/Three-Phase Parallel RLC Load  LConnTagsString=A|B|C  Configuration=Y (grounded)  NominalVoltage=(330000)*1  Vabc=[1e3 1e3 1e3]  Vabcp=[1e3 1e3 1e3]  NominalFrequency=50  UnbalancedPower=off  ActivePower=0  InductivePower=comp(7,3)*1e6  CapacitivePower=comp(7,4)*1e6  Pabc=[10e3 9e3 11e3]  QLabc=[100 90 110]  QCabc=[100 90 110]  Pabcp=[10e3 9e3 11e3]  QLabcp=[100 90 110]  QCabcp=[100 90 110]  Measurements=None  LoadType=constant Z
  Comp8-416 : powerlib/Elements/Three-Phase Parallel RLC Load  LConnTagsString=A|B|C  Configuration=Y (grounded)  NominalVoltage=(330000)*1  Vabc=[1e3 1e3 1e3]  Vabcp=[1e3 1e3 1e3]  NominalFrequency=50  UnbalancedPower=off  ActivePower=0  InductivePower=comp(8,3)*1e6  CapacitivePower=comp(8,4)*1e6  Pabc=[10e3 9e3 11e3]  QLabc=[100 90 110]  QCabc=[100 90 110]  Pabcp=[10e3 9e3 11e3]  QLabcp=[100 90 110]  QCabcp=[100 90 110]  Measurements=None  LoadType=constant Z
  Demux{,1..4} (5 alike) : Demux  Outputs=2
  Dist206 : Subsystem
  Dist212 : Subsystem
  Dist307 : Subsystem
  Dist410 : Subsystem
  Dist411 : Subsystem
  Dist508 : Subsystem
  G201_BPS : Subsystem
  G202_EPS : Subsystem
  G203_VPS : Subsystem
  G204_MPS : Subsystem
  G301_LPS : Subsystem
  G302_YPS : Subsystem
  G401_TPS : Subsystem
  G404_GPS : Subsystem
  G501_NPS : Subsystem
  G503_PPS : Subsystem
  Ground{,1..14} (15 alike) : powerlib/Elements/Ground  LConnTagsString=a
  INV102 : Library/INV  fn=50  Ub=15e3  Pref=Pinit(1)  ang=thetavsc0(1)  K2=Kvsc(1,1)  K1=Kvsc(2,1)
  INV208 : Library/INV  fn=50  Ub=20e3  Pref=Pinit(2)  ang=thetavsc0(2)  K2=Kvsc(1,2)  K1=Kvsc(2,2)
  INV212 : Library/INV  fn=50  Ub=20e3  Pref=Pinit(3)  ang=thetavsc0(3)  K2=Kvsc(1,3)  K1=Kvsc(2,3)
  INV215 : Library/INV  fn=50  Ub=20e3  Pref=Pinit(4)  ang=thetavsc0(4)  K2=Kvsc(1,4)  K1=Kvsc(2,4)
  INV216 : Library/INV  fn=50  Ub=20e3  Pref=Pinit(5)  ang=thetavsc0(5)  K2=Kvsc(1,5)  K1=Kvsc(2,5)
  INV308 : Library/INV  fn=50  Ub=20e3  Pref=Pinit(6)  ang=thetavsc0(6)  K2=Kvsc(1,6)  K1=Kvsc(2,6)
  INV309 : Library/INV  fn=50  Ub=15e3  Pref=Pinit(7)  ang=thetavsc0(7)  K2=Kvsc(1,7)  K1=Kvsc(2,7)
  INV312 : Library/INV  fn=50  Ub=20e3  Pref=Pinit(8)  ang=thetavsc0(8)  K2=Kvsc(1,8)  K1=Kvsc(2,8)
  INV314 : Library/INV  fn=50  Ub=20e3  Pref=Pinit(9)  ang=thetavsc0(9)  K2=Kvsc(1,9)  K1=Kvsc(2,9)
  INV403 : Library/INV  fn=50  Ub=20e3  Pref=Pinit(10)  ang=thetavsc0(10)  K2=Kvsc(1,10)  K1=Kvsc(2,10)
  INV405 : Library/INV  fn=50  Ub=20e3  Pref=Pinit(11)  ang=thetavsc0(11)  K2=Kvsc(1,11)  K1=Kvsc(2,11)
  INV410 : Library/INV  fn=50  Ub=20e3  Pref=Pinit(12)  ang=thetavsc0(12)  K2=Kvsc(1,12)  K1=Kvsc(2,12)
  INV502 : Library/INV  fn=50  Ub=20e3  Pref=Pinit(13)  ang=thetavsc0(13)  K2=Kvsc(1,13)  K1=Kvsc(2,13)
  INV504 : Library/INV  fn=50  Ub=20e3  Pref=Pinit(14)  ang=thetavsc0(14)  K2=Kvsc(1,14)  K1=Kvsc(2,14)
  INV508 : Library/INV  fn=50  Ub=15e3  Pref=Pinit(15)  ang=thetavsc0(15)  K2=Kvsc(1,15)  K1=Kvsc(2,15)
  L-1-1 : powerlib/Elements/Three-Phase PI Section Line  LConnTagsString=a|b|c  RConnTagsString=A|B|C  Frequency=50  Resistances="[ line(1,3)  line(1,3)*3]"  Inductances="[ line(1,4)  line(1,4)*3]"  Capacitances="[ line(1,5)  line(1,5)/3]"  Length=1
      settings: SourceProductName=Simscape Power Systems
  L-1-2 : powerlib/Elements/Three-Phase PI Section Line  LConnTagsString=a|b|c  RConnTagsString=A|B|C  Frequency=50  Resistances="[ line(1,3)  line(1,3)*3]"  Inductances="[ line(1,4)  line(1,4)*3]"  Capacitances="[ line(1,5)  line(1,5)/3]"  Length=1
      settings: SourceProductName=Simscape Power Systems
  L-10-1 : powerlib/Elements/Three-Phase PI Section Line  LConnTagsString=a|b|c  RConnTagsString=A|B|C  Frequency=50  Resistances="[ line(10,3)  line(10,3)*3]"  Inductances="[ line(10,4)  line(10,4)*3]"  Capacitances="[ line(10,5)  line(10,5)/3]"  Length=1
      settings: SourceProductName=Simscape Power Systems
  L-10-2 : powerlib/Elements/Three-Phase PI Section Line  LConnTagsString=a|b|c  RConnTagsString=A|B|C  Frequency=50  Resistances="[ line(10,3)  line(10,3)*3]"  Inductances="[ line(10,4)  line(10,4)*3]"  Capacitances="[ line(10,5)  line(10,5)/3]"  Length=1
      settings: SourceProductName=Simscape Power Systems
  L-11 : powerlib/Elements/Three-Phase PI Section Line  LConnTagsString=a|b|c  RConnTagsString=A|B|C  Frequency=50  Resistances="[ line(11,3)  line(11,3)*3]"  Inductances="[ line(11,4)  line(11,4)*3]"  Capacitances="[ line(11,5)  line(11,5)/3]"  Length=1
      settings: SourceProductName=Simscape Power Systems
  L-12-1 : powerlib/Elements/Three-Phase PI Section Line  LConnTagsString=a|b|c  RConnTagsString=A|B|C  Frequency=50  Resistances="[ line(12,3)  line(12,3)*3]"  Inductances="[ line(12,4)  line(12,4)*3]"  Capacitances="[ line(12,5)  line(12,5)/3]"  Length=1
      settings: SourceProductName=Simscape Power Systems
  L-12-2 : powerlib/Elements/Three-Phase PI Section Line  LConnTagsString=a|b|c  RConnTagsString=A|B|C  Frequency=50  Resistances="[ line(12,3)  line(12,3)*3]"  Inductances="[ line(12,4)  line(12,4)*3]"  Capacitances="[ line(12,5)  line(12,5)/3]"  Length=1
      settings: SourceProductName=Simscape Power Systems
  L-12-3 : powerlib/Elements/Three-Phase PI Section Line  LConnTagsString=a|b|c  RConnTagsString=A|B|C  Frequency=50  Resistances="[ line(12,3)  line(12,3)*3]"  Inductances="[ line(12,4)  line(12,4)*3]"  Capacitances="[ line(12,5)  line(12,5)/3]"  Length=1
      settings: SourceProductName=Simscape Power Systems
  L-13 : powerlib/Elements/Three-Phase PI Section Line  LConnTagsString=a|b|c  RConnTagsString=A|B|C  Frequency=50  Resistances="[ line(13,3)  line(13,3)*3]"  Inductances="[ line(13,4)  line(13,4)*3]"  Capacitances="[ line(13,5)  line(13,5)/3]"  Length=1
      settings: SourceProductName=Simscape Power Systems
  L-14-1 : powerlib/Elements/Three-Phase PI Section Line  LConnTagsString=a|b|c  RConnTagsString=A|B|C  Frequency=50  Resistances="[ line(14,3)  line(14,3)*3]"  Inductances="[ line(14,4)  line(14,4)*3]"  Capacitances="[ line(14,5)  line(14,5)/3]"  Length=1
      settings: SourceProductName=Simscape Power Systems
  L-14-2 : powerlib/Elements/Three-Phase PI Section Line  LConnTagsString=a|b|c  RConnTagsString=A|B|C  Frequency=50  Resistances="[ line(14,3)  line(14,3)*3]"  Inductances="[ line(14,4)  line(14,4)*3]"  Capacitances="[ line(14,5)  line(14,5)/3]"  Length=1
      settings: SourceProductName=Simscape Power Systems
  L-15-1 : powerlib/Elements/Three-Phase PI Section Line  LConnTagsString=a|b|c  RConnTagsString=A|B|C  Frequency=50  Resistances="[ line(15,3)  line(15,3)*3]"  Inductances="[ line(15,4)  line(15,4)*3]"  Capacitances="[ line(15,5)  line(15,5)/3]"  Length=1
      settings: SourceProductName=Simscape Power Systems
  L-15-2 : powerlib/Elements/Three-Phase PI Section Line  LConnTagsString=a|b|c  RConnTagsString=A|B|C  Frequency=50  Resistances="[ line(15,3)  line(15,3)*3]"  Inductances="[ line(15,4)  line(15,4)*3]"  Capacitances="[ line(15,5)  line(15,5)/3]"  Length=1
      settings: SourceProductName=Simscape Power Systems
  L-16 : powerlib/Elements/Three-Phase PI Section Line  LConnTagsString=a|b|c  RConnTagsString=A|B|C  Frequency=50  Resistances="[ line(16,3)  line(16,3)*3]"  Inductances="[ line(16,4)  line(16,4)*3]"  Capacitances="[ line(16,5)  line(16,5)/3]"  Length=1
      settings: SourceProductName=Simscape Power Systems
  L-17 : powerlib/Elements/Three-Phase PI Section Line  LConnTagsString=a|b|c  RConnTagsString=A|B|C  Frequency=50  Resistances="[ line(17,3)  line(17,3)*3]"  Inductances="[ line(17,4)  line(17,4)*3]"  Capacitances="[ line(17,5)  line(17,5)/3]"  Length=1
      settings: SourceProductName=Simscape Power Systems
  L-18 : powerlib/Elements/Three-Phase PI Section Line  LConnTagsString=a|b|c  RConnTagsString=A|B|C  Frequency=50  Resistances="[ line(18,3)  line(18,3)*3]"  Inductances="[ line(18,4)  line(18,4)*3]"  Capacitances="[ line(18,5)  line(18,5)/3]"  Length=1
      settings: SourceProductName=Simscape Power Systems
  L-19 : powerlib/Elements/Three-Phase PI Section Line  LConnTagsString=a|b|c  RConnTagsString=A|B|C  Frequency=50  Resistances="[ line(19,3)  line(19,3)*3]"  Inductances="[ line(19,4)  line(19,4)*3]"  Capacitances="[ line(19,5)  line(19,5)/3]"  Length=1
      settings: SourceProductName=Simscape Power Systems
  L-2-1 : powerlib/Elements/Three-Phase PI Section Line  LConnTagsString=a|b|c  RConnTagsString=A|B|C  Frequency=50  Resistances="[ line(2,3)  line(2,3)*3]"  Inductances="[ line(2,4)  line(2,4)*3]"  Capacitances="[ line(2,5)  line(2,5)/3]"  Length=1
      settings: SourceProductName=Simscape Power Systems
  L-2-2 : powerlib/Elements/Three-Phase PI Section Line  LConnTagsString=a|b|c  RConnTagsString=A|B|C  Frequency=50  Resistances="[ line(2,3)  line(2,3)*3]"  Inductances="[ line(2,4)  line(2,4)*3]"  Capacitances="[ line(2,5)  line(2,5)/3]"  Length=1
      settings: SourceProductName=Simscape Power Systems
  L-20-1 : powerlib/Elements/Three-Phase PI Section Line  LConnTagsString=a|b|c  RConnTagsString=A|B|C  Frequency=50  Resistances="[ line(20,3)  line(20,3)*3]"  Inductances="[ line(20,4)  line(20,4)*3]"  Capacitances="[ line(20,5)  line(20,5)/3]"  Length=1
      settings: SourceProductName=Simscape Power Systems
  L-20-2 : powerlib/Elements/Three-Phase PI Section Line  LConnTagsString=a|b|c  RConnTagsString=A|B|C  Frequency=50  Resistances="[ line(20,3)  line(20,3)*3]"  Inductances="[ line(20,4)  line(20,4)*3]"  Capacitances="[ line(20,5)  line(20,5)/3]"  Length=1
      settings: SourceProductName=Simscape Power Systems
  L-21-1 : powerlib/Elements/Three-Phase PI Section Line  LConnTagsString=a|b|c  RConnTagsString=A|B|C  Frequency=50  Resistances="[ line(21,3)  line(21,3)*3]"  Inductances="[ line(21,4)  line(21,4)*3]"  Capacitances="[ line(21,5)  line(21,5)/3]"  Length=1
      settings: SourceProductName=Simscape Power Systems
  L-21-2 : powerlib/Elements/Three-Phase PI Section Line  LConnTagsString=a|b|c  RConnTagsString=A|B|C  Frequency=50  Resistances="[ line(21,3)  line(21,3)*3]"  Inductances="[ line(21,4)  line(21,4)*3]"  Capacitances="[ line(21,5)  line(21,5)/3]"  Length=1
      settings: SourceProductName=Simscape Power Systems
  L-22 : powerlib/Elements/Three-Phase PI Section Line  LConnTagsString=a|b|c  RConnTagsString=A|B|C  Frequency=50  Resistances="[ line(22,3)  line(22,3)*3]"  Inductances="[ line(22,4)  line(22,4)*3]"  Capacitances="[ line(22,5)  line(22,5)/3]"  Length=1
      settings: SourceProductName=Simscape Power Systems
  L-23 : powerlib/Elements/Three-Phase PI Section Line  LConnTagsString=a|b|c  RConnTagsString=A|B|C  Frequency=50  Resistances="[ line(23,3)  line(23,3)*3]"  Inductances="[ line(23,4)  line(23,4)*3]"  Capacitances="[ line(23,5)  line(23,5)/3]"  Length=1
      settings: SourceProductName=Simscape Power Systems
  L-24-1 : powerlib/Elements/Three-Phase PI Section Line  LConnTagsString=a|b|c  RConnTagsString=A|B|C  Frequency=50  Resistances="[ line(24,3)  line(24,3)*3]"  Inductances="[ line(24,4)  line(24,4)*3]"  Capacitances="[ line(24,5)  line(24,5)/3]"  Length=1
      settings: SourceProductName=Simscape Power Systems
  L-24-2 : powerlib/Elements/Three-Phase PI Section Line  LConnTagsString=a|b|c  RConnTagsString=A|B|C  Frequency=50  Resistances="[ line(24,3)  line(24,3)*3]"  Inductances="[ line(24,4)  line(24,4)*3]"  Capacitances="[ line(24,5)  line(24,5)/3]"  Length=1
      settings: SourceProductName=Simscape Power Systems
  L-25 : powerlib/Elements/Three-Phase PI Section Line  LConnTagsString=a|b|c  RConnTagsString=A|B|C  Frequency=50  Resistances="[ line(25,3)  line(25,3)*3]"  Inductances="[ line(25,4)  line(25,4)*3]"  Capacitances="[ line(25,5)  line(25,5)/3]"  Length=1
      settings: SourceProductName=Simscape Power Systems
  L-26 : powerlib/Elements/Three-Phase PI Section Line  LConnTagsString=a|b|c  RConnTagsString=A|B|C  Frequency=50  Resistances="[ line(26,3)  line(26,3)*3]"  Inductances="[ line(26,4)  line(26,4)*3]"  Capacitances="[ line(26,5)  line(26,5)/3]"  Length=1
      settings: SourceProductName=Simscape Power Systems
  L-27-1 : powerlib/Elements/Three-Phase PI Section Line  LConnTagsString=a|b|c  RConnTagsString=A|B|C  Frequency=50  Resistances="[ line(27,3)  line(27,3)*3]"  Inductances="[ line(27,4)  line(27,4)*3]"  Capacitances="[ line(27,5)  line(27,5)/3]"  Length=1
      settings: SourceProductName=Simscape Power Systems
  L-27-2 : powerlib/Elements/Three-Phase PI Section Line  LConnTagsString=a|b|c  RConnTagsString=A|B|C  Frequency=50  Resistances="[ line(27,3)  line(27,3)*3]"  Inductances="[ line(27,4)  line(27,4)*3]"  Capacitances="[ line(27,5)  line(27,5)/3]"  Length=1
      settings: SourceProductName=Simscape Power Systems
  L-28 : powerlib/Elements/Three-Phase PI Section Line  LConnTagsString=a|b|c  RConnTagsString=A|B|C  Frequency=50  Resistances="[ line(28,3)  line(28,3)*3]"  Inductances="[ line(28,4)  line(28,4)*3]"  Capacitances="[ line(28,5)  line(28,5)/3]"  Length=1
      settings: SourceProductName=Simscape Power Systems
  L-29-1 : powerlib/Elements/Three-Phase PI Section Line  LConnTagsString=a|b|c  RConnTagsString=A|B|C  Frequency=50  Resistances="[ line(29,3)  line(29,3)*3]"  Inductances="[ line(29,4)  line(29,4)*3]"  Capacitances="[ line(29,5)  line(29,5)/3]"  Length=1
      settings: SourceProductName=Simscape Power Systems
  L-29-2 : powerlib/Elements/Three-Phase PI Section Line  LConnTagsString=a|b|c  RConnTagsString=A|B|C  Frequency=50  Resistances="[ line(29,3)  line(29,3)*3]"  Inductances="[ line(29,4)  line(29,4)*3]"  Capacitances="[ line(29,5)  line(29,5)/3]"  Length=1
      settings: SourceProductName=Simscape Power Systems
  L-3-1 : powerlib/Elements/Three-Phase PI Section Line  LConnTagsString=a|b|c  RConnTagsString=A|B|C  Frequency=50  Resistances="[ line(3,3)  line(3,3)*3]"  Inductances="[ line(3,4)  line(3,4)*3]"  Capacitances="[ line(3,5)  line(3,5)/3]"  Length=1
      settings: SourceProductName=Simscape Power Systems
  L-3-2 : powerlib/Elements/Three-Phase PI Section Line  LConnTagsString=a|b|c  RConnTagsString=A|B|C  Frequency=50  Resistances="[ line(3,3)  line(3,3)*3]"  Inductances="[ line(3,4)  line(3,4)*3]"  Capacitances="[ line(3,5)  line(3,5)/3]"  Length=1
      settings: SourceProductName=Simscape Power Systems
  L-30-1 : powerlib/Elements/Three-Phase PI Section Line  LConnTagsString=a|b|c  RConnTagsString=A|B|C  Frequency=50  Resistances="[ line(30,3)  line(30,3)*3]"  Inductances="[ line(30,4)  line(30,4)*3]"  Capacitances="[ line(30,5)  line(30,5)/3]"  Length=1
      settings: SourceProductName=Simscape Power Systems
  L-30-2 : powerlib/Elements/Three-Phase PI Section Line  LConnTagsString=a|b|c  RConnTagsString=A|B|C  Frequency=50  Resistances="[ line(30,3)  line(30,3)*3]"  Inductances="[ line(30,4)  line(30,4)*3]"  Capacitances="[ line(30,5)  line(30,5)/3]"  Length=1
      settings: SourceProductName=Simscape Power Systems
  L-32 : powerlib/Elements/Three-Phase PI Section Line  LConnTagsString=a|b|c  RConnTagsString=A|B|C  Frequency=50  Resistances="[ line(32,3)  line(32,3)*3]"  Inductances="[ line(32,4)  line(32,4)*3]"  Capacitances="[ line(32,5)  line(32,5)/3]"  Length=1
      settings: SourceProductName=Simscape Power Systems
  L-33 : powerlib/Elements/Three-Phase PI Section Line  LConnTagsString=a|b|c  RConnTagsString=A|B|C  Frequency=50  Resistances="[ line(33,3)  line(33,3)*3]"  Inductances="[ line(33,4)  line(33,4)*3]"  Capacitances="[ line(33,5)  line(33,5)/3]"  Length=1
      settings: SourceProductName=Simscape Power Systems
  L-34-1 : powerlib/Elements/Three-Phase PI Section Line  LConnTagsString=a|b|c  RConnTagsString=A|B|C  Frequency=50  Resistances="[ line(34,3)  line(34,3)*3]"  Inductances="[ line(34,4)  line(34,4)*3]"  Capacitances="[ line(34,5)  line(34,5)/3]"  Length=1
      settings: SourceProductName=Simscape Power Systems
  L-34-2 : powerlib/Elements/Three-Phase PI Section Line  LConnTagsString=a|b|c  RConnTagsString=A|B|C  Frequency=50  Resistances="[ line(34,3)  line(34,3)*3]"  Inductances="[ line(34,4)  line(34,4)*3]"  Capacitances="[ line(34,5)  line(34,5)/3]"  Length=1
      settings: SourceProductName=Simscape Power Systems
  L-35-1 : powerlib/Elements/Three-Phase PI Section Line  LConnTagsString=a|b|c  RConnTagsString=A|B|C  Frequency=50  Resistances="[ line(35,3)  line(35,3)*3]"  Inductances="[ line(35,4)  line(35,4)*3]"  Capacitances="[ line(35,5)  line(35,5)/3]"  Length=1
      settings: SourceProductName=Simscape Power Systems
  L-35-2 : powerlib/Elements/Three-Phase PI Section Line  LConnTagsString=a|b|c  RConnTagsString=A|B|C  Frequency=50  Resistances="[ line(35,3)  line(35,3)*3]"  Inductances="[ line(35,4)  line(35,4)*3]"  Capacitances="[ line(35,5)  line(35,5)/3]"  Length=1
      settings: SourceProductName=Simscape Power Systems
  L-36-1 : powerlib/Elements/Three-Phase PI Section Line  LConnTagsString=a|b|c  RConnTagsString=A|B|C  Frequency=50  Resistances="[ line(36,3)  line(36,3)*3]"  Inductances="[ line(36,4)  line(36,4)*3]"  Capacitances="[ line(36,5)  line(36,5)/3]"  Length=1
      settings: SourceProductName=Simscape Power Systems
  L-37-1 : powerlib/Elements/Three-Phase PI Section Line  LConnTagsString=a|b|c  RConnTagsString=A|B|C  Frequency=50  Resistances="[ line(37,3)  line(37,3)*3]"  Inductances="[ line(37,4)  line(37,4)*3]"  Capacitances="[ line(37,5)  line(37,5)/3]"  Length=1
      settings: SourceProductName=Simscape Power Systems
  L-37-2 : powerlib/Elements/Three-Phase PI Section Line  LConnTagsString=a|b|c  RConnTagsString=A|B|C  Frequency=50  Resistances="[ line(37,3)  line(37,3)*3]"  Inductances="[ line(37,4)  line(37,4)*3]"  Capacitances="[ line(37,5)  line(37,5)/3]"  Length=1
      settings: SourceProductName=Simscape Power Systems
  L-37-3 : powerlib/Elements/Three-Phase PI Section Line  LConnTagsString=a|b|c  RConnTagsString=A|B|C  Frequency=50  Resistances="[ line(37,3)  line(37,3)*3]"  Inductances="[ line(37,4)  line(37,4)*3]"  Capacitances="[ line(37,5)  line(37,5)/3]"  Length=1
      settings: SourceProductName=Simscape Power Systems
  L-38-1 : powerlib/Elements/Three-Phase PI Section Line  LConnTagsString=a|b|c  RConnTagsString=A|B|C  Frequency=50  Resistances="[ line(38,3)  line(38,3)*3]"  Inductances="[ line(38,4)  line(38,4)*3]"  Capacitances="[ line(38,5)  line(38,5)/3]"  Length=1
      settings: SourceProductName=Simscape Power Systems
  L-38-2 : powerlib/Elements/Three-Phase PI Section Line  LConnTagsString=a|b|c  RConnTagsString=A|B|C  Frequency=50  Resistances="[ line(38,3)  line(38,3)*3]"  Inductances="[ line(38,4)  line(38,4)*3]"  Capacitances="[ line(38,5)  line(38,5)/3]"  Length=1
      settings: SourceProductName=Simscape Power Systems
  L-39 : powerlib/Elements/Three-Phase PI Section Line  LConnTagsString=a|b|c  RConnTagsString=A|B|C  Frequency=50  Resistances="[ line(39,3)  line(39,3)*3]"  Inductances="[ line(39,4)  line(39,4)*3]"  Capacitances="[ line(39,5)  line(39,5)/3]"  Length=1
      settings: SourceProductName=Simscape Power Systems
  L-4 : powerlib/Elements/Three-Phase PI Section Line  LConnTagsString=a|b|c  RConnTagsString=A|B|C  Frequency=50  Resistances="[ line(4,3)  line(4,3)*3]"  Inductances="[ line(4,4)  line(4,4)*3]"  Capacitances="[ line(4,5)  line(4,5)/3]"  Length=1
      settings: SourceProductName=Simscape Power Systems
  L-40-1 : powerlib/Elements/Three-Phase PI Section Line  LConnTagsString=a|b|c  RConnTagsString=A|B|C  Frequency=50  Resistances="[ line(40,3)  line(40,3)*3]"  Inductances="[ line(40,4)  line(40,4)*3]"  Capacitances="[ line(40,5)  line(40,5)/3]"  Length=1
      settings: SourceProductName=Simscape Power Systems
  L-40-2 : powerlib/Elements/Three-Phase PI Section Line  LConnTagsString=a|b|c  RConnTagsString=A|B|C  Frequency=50  Resistances="[ line(40,3)  line(40,3)*3]"  Inductances="[ line(40,4)  line(40,4)*3]"  Capacitances="[ line(40,5)  line(40,5)/3]"  Length=1
      settings: SourceProductName=Simscape Power Systems
  L-41-1 : powerlib/Elements/Three-Phase PI Section Line  LConnTagsString=a|b|c  RConnTagsString=A|B|C  Frequency=50  Resistances="[ line(41,3)  line(41,3)*3]"  Inductances="[ line(41,4)  line(41,4)*3]"  Capacitances="[ line(41,5)  line(41,5)/3]"  Length=1
      settings: SourceProductName=Simscape Power Systems
  L-41-2 : powerlib/Elements/Three-Phase PI Section Line  LConnTagsString=a|b|c  RConnTagsString=A|B|C  Frequency=50  Resistances="[ line(41,3)  line(41,3)*3]"  Inductances="[ line(41,4)  line(41,4)*3]"  Capacitances="[ line(41,5)  line(41,5)/3]"  Length=1
      settings: SourceProductName=Simscape Power Systems
  L-42 : powerlib/Elements/Three-Phase PI Section Line  LConnTagsString=a|b|c  RConnTagsString=A|B|C  Frequency=50  Resistances="[ line(42,3)  line(42,3)*3]"  Inductances="[ line(42,4)  line(42,4)*3]"  Capacitances="[ line(42,5)  line(42,5)/3]"  Length=1
      settings: SourceProductName=Simscape Power Systems
  L-43-{1..4} (4 alike) : powerlib/Elements/Three-Phase PI Section Line  LConnTagsString=a|b|c  RConnTagsString=A|B|C  Frequency=50  Resistances="[ line(43,3)  line(43,3)*3]"  Inductances="[ line(43,4)  line(43,4)*3]"  Capacitances="[ line(43,5)  line(43,5)/3]"  Length=1
      settings: SourceProductName=Simscape Power Systems
  L-44-1 : powerlib/Elements/Three-Phase PI Section Line  LConnTagsString=a|b|c  RConnTagsString=A|B|C  Frequency=50  Resistances="[ line(44,3)  line(44,3)*3]"  Inductances="[ line(44,4)  line(44,4)*3]"  Capacitances="[ line(44,5)  line(44,5)/3]"  Length=1
      settings: SourceProductName=Simscape Power Systems
  L-44-2 : powerlib/Elements/Three-Phase PI Section Line  LConnTagsString=a|b|c  RConnTagsString=A|B|C  Frequency=50  Resistances="[ line(44,3)  line(44,3)*3]"  Inductances="[ line(44,4)  line(44,4)*3]"  Capacitances="[ line(44,5)  line(44,5)/3]"  Length=1
      settings: SourceProductName=Simscape Power Systems
  L-45-1 : powerlib/Elements/Three-Phase PI Section Line  LConnTagsString=a|b|c  RConnTagsString=A|B|C  Frequency=50  Resistances="[ line(45,3)  line(45,3)*3]"  Inductances="[ line(45,4)  line(45,4)*3]"  Capacitances="[ line(45,5)  line(45,5)/3]"  Length=1
      settings: SourceProductName=Simscape Power Systems
  L-45-2 : powerlib/Elements/Three-Phase PI Section Line  LConnTagsString=a|b|c  RConnTagsString=A|B|C  Frequency=50  Resistances="[ line(45,3)  line(45,3)*3]"  Inductances="[ line(45,4)  line(45,4)*3]"  Capacitances="[ line(45,5)  line(45,5)/3]"  Length=1
      settings: SourceProductName=Simscape Power Systems
  L-46-1 : powerlib/Elements/Three-Phase PI Section Line  LConnTagsString=a|b|c  RConnTagsString=A|B|C  Frequency=50  Resistances="[ line(46,3)  line(46,3)*3]"  Inductances="[ line(46,4)  line(46,4)*3]"  Capacitances="[ line(46,5)  line(46,5)/3]"  Length=1
      settings: SourceProductName=Simscape Power Systems
  L-46-2 : powerlib/Elements/Three-Phase PI Section Line  LConnTagsString=a|b|c  RConnTagsString=A|B|C  Frequency=50  Resistances="[ line(46,3)  line(46,3)*3]"  Inductances="[ line(46,4)  line(46,4)*3]"  Capacitances="[ line(46,5)  line(46,5)/3]"  Length=1
      settings: SourceProductName=Simscape Power Systems
  L-47-1 : powerlib/Elements/Three-Phase PI Section Line  LConnTagsString=a|b|c  RConnTagsString=A|B|C  Frequency=50  Resistances="[ line(47,3)  line(47,3)*3]"  Inductances="[ line(47,4)  line(47,4)*3]"  Capacitances="[ line(47,5)  line(47,5)/3]"  Length=1
      settings: SourceProductName=Simscape Power Systems
  L-47-2 : powerlib/Elements/Three-Phase PI Section Line  LConnTagsString=a|b|c  RConnTagsString=A|B|C  Frequency=50  Resistances="[ line(47,3)  line(47,3)*3]"  Inductances="[ line(47,4)  line(47,4)*3]"  Capacitances="[ line(47,5)  line(47,5)/3]"  Length=1
      settings: SourceProductName=Simscape Power Systems
  L-48-1 : powerlib/Elements/Three-Phase PI Section Line  LConnTagsString=a|b|c  RConnTagsString=A|B|C  Frequency=50  Resistances="[ line(48,3)  line(48,3)*3]"  Inductances="[ line(48,4)  line(48,4)*3]"  Capacitances="[ line(48,5)  line(48,5)/3]"  Length=1
      settings: SourceProductName=Simscape Power Systems
  L-48-2 : powerlib/Elements/Three-Phase PI Section Line  LConnTagsString=a|b|c  RConnTagsString=A|B|C  Frequency=50  Resistances="[ line(48,3)  line(48,3)*3]"  Inductances="[ line(48,4)  line(48,4)*3]"  Capacitances="[ line(48,5)  line(48,5)/3]"  Length=1
      settings: SourceProductName=Simscape Power Systems
  L-49-1 : powerlib/Elements/Three-Phase PI Section Line  LConnTagsString=a|b|c  RConnTagsString=A|B|C  Frequency=50  Resistances="[ line(49,3)  line(49,3)*3]"  Inductances="[ line(49,4)  line(49,4)*3]"  Capacitances="[ line(49,5)  line(49,5)/3]"  Length=1
      settings: SourceProductName=Simscape Power Systems
  L-49-2 : powerlib/Elements/Three-Phase PI Section Line  LConnTagsString=a|b|c  RConnTagsString=A|B|C  Frequency=50  Resistances="[ line(49,3)  line(49,3)*3]"  Inductances="[ line(49,4)  line(49,4)*3]"  Capacitances="[ line(49,5)  line(49,5)/3]"  Length=1
      settings: SourceProductName=Simscape Power Systems
  L-5-1 : powerlib/Elements/Three-Phase PI Section Line  LConnTagsString=a|b|c  RConnTagsString=A|B|C  Frequency=50  Resistances="[ line(5,3)  line(5,3)*3]"  Inductances="[ line(5,4)  line(5,4)*3]"  Capacitances="[ line(5,5)  line(5,5)/3]"  Length=1
      settings: SourceProductName=Simscape Power Systems
  L-5-2 : powerlib/Elements/Three-Phase PI Section Line  LConnTagsString=a|b|c  RConnTagsString=A|B|C  Frequency=50  Resistances="[ line(5,3)  line(5,3)*3]"  Inductances="[ line(5,4)  line(5,4)*3]"  Capacitances="[ line(5,5)  line(5,5)/3]"  Length=1
      settings: SourceProductName=Simscape Power Systems
  L-50-1 : powerlib/Elements/Three-Phase PI Section Line  LConnTagsString=a|b|c  RConnTagsString=A|B|C  Frequency=50  Resistances="[ line(50,3)  line(50,3)*3]"  Inductances="[ line(50,4)  line(50,4)*3]"  Capacitances="[ line(50,5)  line(50,5)/3]"  Length=1
      settings: SourceProductName=Simscape Power Systems
  L-51 : powerlib/Elements/Three-Phase PI Section Line  LConnTagsString=a|b|c  RConnTagsString=A|B|C  Frequency=50  Resistances="[ line(51,3)  line(51,3)*3]"  Inductances="[ line(51,4)  line(51,4)*3]"  Capacitances="[ line(51,5)  line(51,5)/3]"  Length=1
      settings: SourceProductName=Simscape Power Systems
  L-52 : powerlib/Elements/Three-Phase PI Section Line  LConnTagsString=a|b|c  RConnTagsString=A|B|C  Frequency=50  Resistances="[ line(52,3)  line(52,3)*3]"  Inductances="[ line(52,4)  line(52,4)*3]"  Capacitances="[ line(52,5)  line(52,5)/3]"  Length=1
      settings: SourceProductName=Simscape Power Systems
  L-53 : powerlib/Elements/Three-Phase PI Section Line  LConnTagsString=a|b|c  RConnTagsString=A|B|C  Frequency=50  Resistances="[ line(53,3)  line(53,3)*3]"  Inductances="[ line(53,4)  line(53,4)*3]"  Capacitances="[ line(53,5)  line(53,5)/3]"  Length=1
      settings: SourceProductName=Simscape Power Systems
  L-54 : powerlib/Elements/Three-Phase PI Section Line  LConnTagsString=a|b|c  RConnTagsString=A|B|C  Frequency=50  Resistances=[ line(54,3) line(54,3)*3]  Inductances=[ line(54,4) line(54,4)*3]  Capacitances=[ line(54,5) line(54,5)/3]  Length=1
      settings: SourceProductName=Simscape Power Systems
  L-55-1 : powerlib/Elements/Three-Phase PI Section Line  LConnTagsString=a|b|c  RConnTagsString=A|B|C  Frequency=50  Resistances=[ line(55,3) line(55,3)*3]  Inductances="[ line(55,4)  line(55,4)*3]"  Capacitances="[line(55,5)  line(55,5)/3]"  Length=1
      settings: SourceProductName=Simscape Power Systems
  L-55-2 : powerlib/Elements/Three-Phase PI Section Line  LConnTagsString=a|b|c  RConnTagsString=A|B|C  Frequency=50  Resistances=[ line(55,3) line(55,3)*3]  Inductances="[ line(55,4)  line(55,4)*3]"  Capacitances="[line(55,5)  line(55,5)/3]"  Length=1
      settings: SourceProductName=Simscape Power Systems
  L-6-1 : powerlib/Elements/Three-Phase PI Section Line  LConnTagsString=a|b|c  RConnTagsString=A|B|C  Frequency=50  Resistances="[ line(6,3)  line(6,3)*3]"  Inductances="[ line(6,4)  line(6,4)*3]"  Capacitances="[ line(6,5)  line(6,5)/3]"  Length=1
      settings: SourceProductName=Simscape Power Systems
  L-6-2 : powerlib/Elements/Three-Phase PI Section Line  LConnTagsString=a|b|c  RConnTagsString=A|B|C  Frequency=50  Resistances="[ line(6,3)  line(6,3)*3]"  Inductances="[ line(6,4)  line(6,4)*3]"  Capacitances="[ line(6,5)  line(6,5)/3]"  Length=1
      settings: SourceProductName=Simscape Power Systems
  L-7-1 : powerlib/Elements/Three-Phase PI Section Line  LConnTagsString=a|b|c  RConnTagsString=A|B|C  Frequency=50  Resistances="[ line(7,3)  line(7,3)*3]"  Inductances="[ line(7,4)  line(7,4)*3]"  Capacitances="[ line(7,5)  line(7,5)/3]"  Length=1
      settings: SourceProductName=Simscape Power Systems
  L-7-2 : powerlib/Elements/Three-Phase PI Section Line  LConnTagsString=a|b|c  RConnTagsString=A|B|C  Frequency=50  Resistances="[ line(7,3)  line(7,3)*3]"  Inductances="[ line(7,4)  line(7,4)*3]"  Capacitances="[ line(7,5)  line(7,5)/3]"  Length=1
      settings: SourceProductName=Simscape Power Systems
  L-8-1 : powerlib/Elements/Three-Phase PI Section Line  LConnTagsString=a|b|c  RConnTagsString=A|B|C  Frequency=50  Resistances="[ line(8,3)  line(8,3)*3]"  Inductances="[ line(8,4)  line(8,4)*3]"  Capacitances="[ line(8,5)  line(8,5)/3]"  Length=1
      settings: SourceProductName=Simscape Power Systems
  L-8-2 : powerlib/Elements/Three-Phase PI Section Line  LConnTagsString=a|b|c  RConnTagsString=A|B|C  Frequency=50  Resistances="[ line(8,3)  line(8,3)*3]"  Inductances="[ line(8,4)  line(8,4)*3]"  Capacitances="[ line(8,5)  line(8,5)/3]"  Length=1
      settings: SourceProductName=Simscape Power Systems
  L-9-1 : powerlib/Elements/Three-Phase PI Section Line  LConnTagsString=a|b|c  RConnTagsString=A|B|C  Frequency=50  Resistances="[ line(9,3)  line(9,3)*3]"  Inductances="[ line(9,4)  line(9,4)*3]"  Capacitances="[ line(9,5)  line(9,5)/3]"  Length=1
      settings: SourceProductName=Simscape Power Systems
  L-9-2 : powerlib/Elements/Three-Phase PI Section Line  LConnTagsString=a|b|c  RConnTagsString=A|B|C  Frequency=50  Resistances="[ line(9,3)  line(9,3)*3]"  Inductances="[ line(9,4)  line(9,4)*3]"  Capacitances="[ line(9,5)  line(9,5)/3]"  Length=1
      settings: SourceProductName=Simscape Power Systems
  Load Flow Bus1 : powerlib/Measurements/Load Flow Bus  LConnTagsString=a  Phases=single  Connectors=on one side  ID=B403_vsw  Vbase=20e3  Vref=1  Vangle=0  VLF=0.9972  VLFb=1  VLFc=1  angleLF=23.58  angleLFb=0  angleLFc=0
      settings: AttributesFormatString=%<ID>\n%<Vbase>V\n%<VLF>pu\n%<angleLF>deg.  SourceProductName=Simscape Power Systems
  Load Flow Bus10 : powerlib/Measurements/Load Flow Bus  LConnTagsString=a  Phases=single  Connectors=on one side  ID=B301  Vbase=20e3  Vref=1  Vangle=0  VLF=1  VLFb=1  VLFc=1  angleLF=-10.04  angleLFb=0  angleLFc=0
      settings: AttributesFormatString=%<ID>\n%<Vbase>V\n%<VLF>pu\n%<angleLF>deg.  SourceProductName=Simscape Power Systems
  Load Flow Bus11 : powerlib/Measurements/Load Flow Bus  LConnTagsString=a  Phases=single  Connectors=on one side  ID=B302  Vbase=20e3  Vref=1  Vangle=0  VLF=1  VLFb=1  VLFc=1  angleLF=-18.96  angleLFb=0  angleLFc=0
      settings: AttributesFormatString=%<ID>\n%<Vbase>V\n%<VLF>pu\n%<angleLF>deg.  SourceProductName=Simscape Power Systems
  Load Flow Bus12 : powerlib/Measurements/Load Flow Bus  LConnTagsString=a  Phases=single  Connectors=on one side  ID=B503  Vbase=15e3  Vref=1  Vangle=0  VLF=1  VLFb=1  VLFc=1  angleLF=-38.47  angleLFb=0  angleLFc=0
      settings: AttributesFormatString=%<ID>\n%<Vbase>V\n%<VLF>pu\n%<angleLF>deg.  SourceProductName=Simscape Power Systems
  Load Flow Bus13 : powerlib/Measurements/Load Flow Bus  LConnTagsString=a  Phases=single  Connectors=on one side  ID=B502  Vbase=15e3  Vref=1  Vangle=0  VLF=0.9992  VLFb=1  VLFc=1  angleLF=-2.878  angleLFb=0  angleLFc=0
      settings: AttributesFormatString=%<ID>\n%<Vbase>V\n%<VLF>pu\n%<angleLF>deg.  SourceProductName=Simscape Power Systems
  Load Flow Bus14 : powerlib/Measurements/Load Flow Bus  LConnTagsString=a  Phases=single  Connectors=on one side  ID=B501  Vbase=20e3  Vref=1  Vangle=0  VLF=1  VLFb=1  VLFc=1  angleLF=-34.56  angleLFb=0  angleLFc=0
      settings: AttributesFormatString=%<ID>\n%<Vbase>V\n%<VLF>pu\n%<angleLF>deg.  SourceProductName=Simscape Power Systems
  Load Flow Bus15 : powerlib/Measurements/Load Flow Bus  LConnTagsString=a  Phases=single  Connectors=on one side  ID=B403  Vbase=20e3  Vref=1  Vangle=0  VLF=0.9972  VLFb=1  VLFc=1  angleLF=23.58  angleLFb=0  angleLFc=0
      settings: AttributesFormatString=%<ID>\n%<Vbase>V\n%<VLF>pu\n%<angleLF>deg.  SourceProductName=Simscape Power Systems
  Load Flow Bus16 : powerlib/Measurements/Load Flow Bus  LConnTagsString=a  Phases=single  Connectors=on one side  ID=B410_vsw  Vbase=20e3  Vref=1  Vangle=0  VLF=1  VLFb=1  VLFc=1  angleLF=2.825  angleLFb=0  angleLFc=0
      settings: AttributesFormatString=%<ID>\n%<Vbase>V\n%<VLF>pu\n%<angleLF>deg.  SourceProductName=Simscape Power Systems
  Load Flow Bus17 : powerlib/Measurements/Load Flow Bus  LConnTagsString=a  Phases=single  Connectors=on one side  ID=B504_vsw  Vbase=20e3  Vref=1  Vangle=0  VLF=1  VLFb=1  VLFc=1  angleLF=-12.45  angleLFb=0  angleLFc=0
      settings: AttributesFormatString=%<ID>\n%<Vbase>V\n%<VLF>pu\n%<angleLF>deg.  SourceProductName=Simscape Power Systems
  Load Flow Bus18 : powerlib/Measurements/Load Flow Bus  LConnTagsString=a  Phases=single  Connectors=on one side  ID=B502_vsw  Vbase=20e3  Vref=1  Vangle=0  VLF=1  VLFb=1  VLFc=1  angleLF=-12.71  angleLFb=0  angleLFc=0
      settings: AttributesFormatString=%<ID>\n%<Vbase>V\n%<VLF>pu\n%<angleLF>deg.  SourceProductName=Simscape Power Systems
  Load Flow Bus19 : powerlib/Measurements/Load Flow Bus  LConnTagsString=a  Phases=single  Connectors=on one side  ID=B508_vsw  Vbase=15e3  Vref=1  Vangle=0  VLF=1  VLFb=1  VLFc=1  angleLF=-14.76  angleLFb=0  angleLFc=0
      settings: AttributesFormatString=%<ID>\n%<Vbase>V\n%<VLF>pu\n%<angleLF>deg.  SourceProductName=Simscape Power Systems
  Load Flow Bus2 : powerlib/Measurements/Load Flow Bus  LConnTagsString=a  Phases=single  Connectors=on one side  ID=B404  Vbase=20e3  Vref=1  Vangle=0  VLF=1  VLFb=1  VLFc=1  angleLF=-13.1  angleLFb=0  angleLFc=0
      settings: AttributesFormatString=%<ID>\n%<Vbase>V\n%<VLF>pu\n%<angleLF>deg.  SourceProductName=Simscape Power Systems
  Load Flow Bus20 : powerlib/Measurements/Load Flow Bus  LConnTagsString=a  Phases=single  Connectors=on one side  ID=B308_vsw  Vbase=20e3  Vref=1  Vangle=0  VLF=1  VLFb=1  VLFc=1  angleLF=-6.338  angleLFb=0  angleLFc=0
      settings: AttributesFormatString=%<ID>\n%<Vbase>V\n%<VLF>pu\n%<angleLF>deg.  SourceProductName=Simscape Power Systems
  Load Flow Bus21 : powerlib/Measurements/Load Flow Bus  LConnTagsString=a  Phases=single  Connectors=on one side  ID=B314_vsw  Vbase=20e3  Vref=1  Vangle=0  VLF=1  VLFb=1  VLFc=1  angleLF=-1.099  angleLFb=0  angleLFc=0
      settings: AttributesFormatString=%<ID>\n%<Vbase>V\n%<VLF>pu\n%<angleLF>deg.  SourceProductName=Simscape Power Systems
  Load Flow Bus22 : powerlib/Measurements/Load Flow Bus  LConnTagsString=a  Phases=single  Connectors=on one side  ID=B312_vsw  Vbase=20e3  Vref=1  Vangle=0  VLF=1  VLFb=1  VLFc=1  angleLF=3.684  angleLFb=0  angleLFc=0
      settings: AttributesFormatString=%<ID>\n%<Vbase>V\n%<VLF>pu\n%<angleLF>deg.  SourceProductName=Simscape Power Systems
  Load Flow Bus23 : powerlib/Measurements/Load Flow Bus  LConnTagsString=a  Phases=single  Connectors=on one side  ID=B309_vsw  Vbase=15e3  Vref=1  Vangle=0  VLF=1  VLFb=1  VLFc=1  angleLF=4.793  angleLFb=0  angleLFc=0
      settings: AttributesFormatString=%<ID>\n%<Vbase>V\n%<VLF>pu\n%<angleLF>deg.  SourceProductName=Simscape Power Systems
  Load Flow Bus24 : powerlib/Measurements/Load Flow Bus  LConnTagsString=a  Phases=single  Connectors=on one side  ID=B102_vsw  Vbase=15e3  Vref=1  Vangle=0  VLF=1  VLFb=1  VLFc=1  angleLF=6.617  angleLFb=0  angleLFc=0
      settings: AttributesFormatString=%<ID>\n%<Vbase>V\n%<VLF>pu\n%<angleLF>deg.  SourceProductName=Simscape Power Systems
  Load Flow Bus25 : powerlib/Measurements/Load Flow Bus  LConnTagsString=a  Phases=single  Connectors=on one side  ID=B216_vsw  Vbase=20e3  Vref=1  Vangle=0  VLF=1  VLFb=1  VLFc=1  angleLF=14.02  angleLFb=0  angleLFc=0
      settings: AttributesFormatString=%<ID>\n%<Vbase>V\n%<VLF>pu\n%<angleLF>deg.  SourceProductName=Simscape Power Systems
  Load Flow Bus26 : powerlib/Measurements/Load Flow Bus  LConnTagsString=a  Phases=single  Connectors=on one side  ID=B215_vsw  Vbase=20e3  Vref=1  Vangle=0  VLF=1  VLFb=1  VLFc=1  angleLF=23.87  angleLFb=0  angleLFc=0
      settings: AttributesFormatString=%<ID>\n%<Vbase>V\n%<VLF>pu\n%<angleLF>deg.  SourceProductName=Simscape Power Systems
  Load Flow Bus27 : powerlib/Measurements/Load Flow Bus  LConnTagsString=a  Phases=single  Connectors=on one side  ID=B212_vsw  Vbase=20e3  Vref=1  Vangle=0  VLF=1  VLFb=1  VLFc=1  angleLF=15.52  angleLFb=0  angleLFc=0
      settings: AttributesFormatString=%<ID>\n%<Vbase>V\n%<VLF>pu\n%<angleLF>deg.  SourceProductName=Simscape Power Systems
  Load Flow Bus28 : powerlib/Measurements/Load Flow Bus  LConnTagsString=a  Phases=single  Connectors=on one side  ID=B208_vsw  Vbase=20e3  Vref=1  Vangle=0  VLF=1  VLFb=1  VLFc=1  angleLF=21.27  angleLFb=0  angleLFc=0
      settings: AttributesFormatString=%<ID>\n%<Vbase>V\n%<VLF>pu\n%<angleLF>deg.  SourceProductName=Simscape Power Systems
  Load Flow Bus29 : powerlib/Measurements/Load Flow Bus  LConnTagsString=a  Phases=single  Connectors=on one side  ID=B405_vsw  Vbase=20e3  Vref=1  Vangle=0  VLF=0.9972  VLFb=1  VLFc=1  angleLF=23.58  angleLFb=0  angleLFc=0
      settings: AttributesFormatString=%<ID>\n%<Vbase>V\n%<VLF>pu\n%<angleLF>deg.  SourceProductName=Simscape Power Systems
  Load Flow Bus3 : powerlib/Measurements/Load Flow Bus  LConnTagsString=a  Phases=single  Connectors=on one side  ID=B402  Vbase=20e3  Vref=1  Vangle=0  VLF=0.9966  VLFb=1  VLFc=1  angleLF=23.92  angleLFb=0  angleLFc=0
      settings: AttributesFormatString=%<ID>\n%<Vbase>V\n%<VLF>pu\n%<angleLF>deg.  SourceProductName=Simscape Power Systems
  Load Flow Bus4 : powerlib/Measurements/Load Flow Bus  LConnTagsString=a  Phases=single  Connectors=on one side  ID=B401  Vbase=20e3  Vref=1  Vangle=0  VLF=1  VLFb=1  VLFc=1  angleLF=-21.06  angleLFb=0  angleLFc=0
      settings: AttributesFormatString=%<ID>\n%<Vbase>V\n%<VLF>pu\n%<angleLF>deg.  SourceProductName=Simscape Power Systems
  Load Flow Bus5 : powerlib/Measurements/Load Flow Bus  LConnTagsString=a  Phases=single  Connectors=on one side  ID=B203  Vbase=20e3  Vref=1  Vangle=0  VLF=1  VLFb=1  VLFc=1  angleLF=-0.543  angleLFb=0  angleLFc=0
      settings: AttributesFormatString=%<ID>\n%<Vbase>V\n%<VLF>pu\n%<angleLF>deg.  SourceProductName=Simscape Power Systems
  Load Flow Bus6 : powerlib/Measurements/Load Flow Bus  LConnTagsString=a  Phases=single  Connectors=on one side  ID=B201  Vbase=20e3  Vref=1  Vangle=0  VLF=1  VLFb=1  VLFc=1  angleLF=3.923  angleLFb=0  angleLFc=0
      settings: AttributesFormatString=%<ID>\n%<Vbase>V\n%<VLF>pu\n%<angleLF>deg.  SourceProductName=Simscape Power Systems
  Load Flow Bus7 : powerlib/Measurements/Load Flow Bus  LConnTagsString=a  Phases=single  Connectors=on one side  ID=B202  Vbase=20e3  Vref=1  Vangle=0  VLF=1  VLFb=1  VLFc=1  angleLF=-0.2053  angleLFb=0  angleLFc=0
      settings: AttributesFormatString=%<ID>\n%<Vbase>V\n%<VLF>pu\n%<angleLF>deg.  SourceProductName=Simscape Power Systems
  Load Flow Bus8 : powerlib/Measurements/Load Flow Bus  LConnTagsString=a  Phases=single  Connectors=on one side  ID=B204  Vbase=20e3  Vref=1  Vangle=0  VLF=1  VLFb=1  VLFc=1  angleLF=0  angleLFb=0  angleLFc=0
      settings: AttributesFormatString=%<ID>\n%<Vbase>V\n%<VLF>pu\n%<angleLF>deg.  SourceProductName=Simscape Power Systems
  Load Flow Bus9 : powerlib/Measurements/Load Flow Bus  LConnTagsString=a  Phases=single  Connectors=on one side  ID=B101  Vbase=15e3  Vref=1  Vangle=0  VLF=1.083  VLFb=1  VLFc=1  angleLF=6.603  angleLFb=0  angleLFc=0
      settings: AttributesFormatString=%<ID>\n%<Vbase>V\n%<VLF>pu\n%<angleLF>deg.  SourceProductName=Simscape Power Systems
  Load1 : powerlib/Elements/Three-Phase Parallel RLC Load  LConnTagsString=A|B|C  Configuration=Y (grounded)  NominalVoltage=(356540)*1.00295  Vabc=[1e3 1e3 1e3]  Vabcp=[1e3 1e3 1e3]  NominalFrequency=50  UnbalancedPower=off  ActivePower=load_mag(1,2)*1e6  InductivePower=load_mag(1,3)*1e6  CapacitivePower=0  Pabc=[10e3 9e3 11e3]  QLabc=[100 90 110]  QCabc=[100 90 110]  Pabcp=[10e3 9e3 11e3]  QLabcp=[100 90 110]  QCabcp=[100 90 110]  Measurements=None  LoadType=constant PQ
  Load10 : powerlib/Elements/Three-Phase Parallel RLC Load  LConnTagsString=A|B|C  Configuration=Y (grounded)  NominalVoltage=(346286)*1.00201  Vabc=[1e3 1e3 1e3]  Vabcp=[1e3 1e3 1e3]  NominalFrequency=50  UnbalancedPower=off  ActivePower=load_mag(10,2)*1e6  InductivePower=load_mag(10,3)*1e6  CapacitivePower=0  Pabc=[10e3 9e3 11e3]  QLabc=[100 90 110]  QCabc=[100 90 110]  Pabcp=[10e3 9e3 11e3]  QLabcp=[100 90 110]  QCabcp=[100 90 110]  Measurements=None  LoadType=constant PQ
  Load11 : powerlib/Elements/Three-Phase Parallel RLC Load  LConnTagsString=A|B|C  Configuration=Y (grounded)  NominalVoltage=(511149)*1.0019  Vabc=[1e3 1e3 1e3]  Vabcp=[1e3 1e3 1e3]  NominalFrequency=50  UnbalancedPower=off  ActivePower=load_mag(11,2)*1e6  InductivePower=load_mag(11,3)*1e6  CapacitivePower=0  Pabc=[10e3 9e3 11e3]  QLabc=[100 90 110]  QCabc=[100 90 110]  Pabcp=[10e3 9e3 11e3]  QLabcp=[100 90 110]  QCabcp=[100 90 110]  Measurements=None  LoadType=constant PQ
  Load12 : powerlib/Elements/Three-Phase Parallel RLC Load  LConnTagsString=A|B|C  Configuration=Y (grounded)  NominalVoltage=(512503)*1.00192  Vabc=[1e3 1e3 1e3]  Vabcp=[1e3 1e3 1e3]  NominalFrequency=50  UnbalancedPower=off  ActivePower=load_mag(12,2)*1e6  InductivePower=load_mag(12,3)*1e6  CapacitivePower=0  Pabc=[10e3 9e3 11e3]  QLabc=[100 90 110]  QCabc=[100 90 110]  Pabcp=[10e3 9e3 11e3]  QLabcp=[100 90 110]  QCabcp=[100 90 110]  Measurements=None  LoadType=constant PQ
  Load13 : powerlib/Elements/Three-Phase Parallel RLC Load  LConnTagsString=A|B|C  Configuration=Y (grounded)  NominalVoltage=(529566)*1.00301  Vabc=[1e3 1e3 1e3]  Vabcp=[1e3 1e3 1e3]  NominalFrequency=50  UnbalancedPower=off  ActivePower=load_mag(13,2)*1e6  InductivePower=load_mag(13,3)*1e6  CapacitivePower=0  Pabc=[10e3 9e3 11e3]  QLabc=[100 90 110]  QCabc=[100 90 110]  Pabcp=[10e3 9e3 11e3]  QLabcp=[100 90 110]  QCabcp=[100 90 110]  Measurements=None  LoadType=constant PQ
  Load14 : powerlib/Elements/Three-Phase Parallel RLC Load  LConnTagsString=A|B|C  Configuration=Y (grounded)  NominalVoltage=(357825)*1.00308  Vabc=[1e3 1e3 1e3]  Vabcp=[1e3 1e3 1e3]  NominalFrequency=50  UnbalancedPower=off  ActivePower=load_mag(14,2)*1e6  InductivePower=load_mag(14,3)*1e6  CapacitivePower=0  Pabc=[10e3 9e3 11e3]  QLabc=[100 90 110]  QCabc=[100 90 110]  Pabcp=[10e3 9e3 11e3]  QLabcp=[100 90 110]  QCabcp=[100 90 110]  Measurements=None  LoadType=constant PQ
  Load15 : powerlib/Elements/Three-Phase Parallel RLC Load  LConnTagsString=A|B|C  Configuration=Y (grounded)  NominalVoltage=(220026)*1.00158  Vabc=[1e3 1e3 1e3]  Vabcp=[1e3 1e3 1e3]  NominalFrequency=50  UnbalancedPower=off  ActivePower=load_mag(15,2)*1e6  InductivePower=load_mag(15,3)*1e6  CapacitivePower=0  Pabc=[10e3 9e3 11e3]  QLabc=[100 90 110]  QCabc=[100 90 110]  Pabcp=[10e3 9e3 11e3]  QLabcp=[100 90 110]  QCabcp=[100 90 110]  Measurements=None  LoadType=constant PQ
  Load16 : powerlib/Elements/Three-Phase Parallel RLC Load  LConnTagsString=A|B|C  Configuration=Y (grounded)  NominalVoltage=(218962)*1.00201  Vabc=[1e3 1e3 1e3]  Vabcp=[1e3 1e3 1e3]  NominalFrequency=50  UnbalancedPower=off  ActivePower=load_mag(16,2)*1e6  InductivePower=load_mag(16,3)*1e6  CapacitivePower=0  Pabc=[10e3 9e3 11e3]  QLabc=[100 90 110]  QCabc=[100 90 110]  Pabcp=[10e3 9e3 11e3]  QLabcp=[100 90 110]  QCabcp=[100 90 110]  Measurements=None  LoadType=constant PQ
  Load17 : powerlib/Elements/Three-Phase Parallel RLC Load  LConnTagsString=A|B|C  Configuration=Y (grounded)  NominalVoltage=(220626)*1.00218  Vabc=[1e3 1e3 1e3]  Vabcp=[1e3 1e3 1e3]  NominalFrequency=50  UnbalancedPower=off  ActivePower=load_mag(17,2)*1e6  InductivePower=load_mag(17,3)*1e6  CapacitivePower=0  Pabc=[10e3 9e3 11e3]  QLabc=[100 90 110]  QCabc=[100 90 110]  Pabcp=[10e3 9e3 11e3]  QLabcp=[100 90 110]  QCabcp=[100 90 110]  Measurements=None  LoadType=constant PQ
  Load18 : powerlib/Elements/Three-Phase Parallel RLC Load  LConnTagsString=A|B|C  Configuration=Y (grounded)  NominalVoltage=(276748)*1.00132  Vabc=[1e3 1e3 1e3]  Vabcp=[1e3 1e3 1e3]  NominalFrequency=50  UnbalancedPower=off  ActivePower=load_mag(18,2)*1e6  InductivePower=load_mag(18,3)*1e6  CapacitivePower=0  Pabc=[10e3 9e3 11e3]  QLabc=[100 90 110]  QCabc=[100 90 110]  Pabcp=[10e3 9e3 11e3]  QLabcp=[100 90 110]  QCabcp=[100 90 110]  Measurements=None  LoadType=constant PQ
  Load19 : powerlib/Elements/Three-Phase Parallel RLC Load  LConnTagsString=A|B|C  Configuration=Y (grounded)  NominalVoltage=(273917)*1.00148  Vabc=[1e3 1e3 1e3]  Vabcp=[1e3 1e3 1e3]  NominalFrequency=50  UnbalancedPower=off  ActivePower=load_mag(19,2)*1e6  InductivePower=load_mag(19,3)*1e6  CapacitivePower=0  Pabc=[10e3 9e3 11e3]  QLabc=[100 90 110]  QCabc=[100 90 110]  Pabcp=[10e3 9e3 11e3]  QLabcp=[100 90 110]  QCabcp=[100 90 110]  Measurements=None  LoadType=constant PQ
  Load2 : powerlib/Elements/Three-Phase Parallel RLC Load  LConnTagsString=A|B|C  Configuration=Y (grounded)  NominalVoltage=(346402)*1.00069  Vabc=[1e3 1e3 1e3]  Vabcp=[1e3 1e3 1e3]  NominalFrequency=50  UnbalancedPower=off  ActivePower=load_mag(2,2)*1e6  InductivePower=load_mag(2,3)*1e6  CapacitivePower=0  Pabc=[10e3 9e3 11e3]  QLabc=[100 90 110]  QCabc=[100 90 110]  Pabcp=[10e3 9e3 11e3]  QLabcp=[100 90 110]  QCabcp=[100 90 110]  Measurements=None  LoadType=constant PQ
  Load20 : powerlib/Elements/Three-Phase Parallel RLC Load  LConnTagsString=A|B|C  Configuration=Y (grounded)  NominalVoltage=(274336)*1.00148  Vabc=[1e3 1e3 1e3]  Vabcp=[1e3 1e3 1e3]  NominalFrequency=50  UnbalancedPower=off  ActivePower=load_mag(20,2)*1e6  InductivePower=load_mag(20,3)*1e6  CapacitivePower=0  Pabc=[10e3 9e3 11e3]  QLabc=[100 90 110]  QCabc=[100 90 110]  Pabcp=[10e3 9e3 11e3]  QLabcp=[100 90 110]  QCabcp=[100 90 110]  Measurements=None  LoadType=constant PQ
  Load21 : powerlib/Elements/Three-Phase Parallel RLC Load  LConnTagsString=A|B|C  Configuration=Y (grounded)  NominalVoltage=(277487)*1.0014  Vabc=[1e3 1e3 1e3]  Vabcp=[1e3 1e3 1e3]  NominalFrequency=50  UnbalancedPower=off  ActivePower=load_mag(21,2)*1e6  InductivePower=load_mag(21,3)*1e6  CapacitivePower=0  Pabc=[10e3 9e3 11e3]  QLabc=[100 90 110]  QCabc=[100 90 110]  Pabcp=[10e3 9e3 11e3]  QLabcp=[100 90 110]  QCabcp=[100 90 110]  Measurements=None  LoadType=constant PQ
  Load22 : powerlib/Elements/Three-Phase Parallel RLC Load  LConnTagsString=A|B|C  Configuration=Y (grounded)  NominalVoltage=(275000)*1.03603  Vabc=[1e3 1e3 1e3]  Vabcp=[1e3 1e3 1e3]  NominalFrequency=50  UnbalancedPower=off  ActivePower=load_mag(22,2)*1e6  InductivePower=load_mag(22,3)*1e6  CapacitivePower=0  Pabc=[10e3 9e3 11e3]  QLabc=[100 90 110]  QCabc=[100 90 110]  Pabcp=[10e3 9e3 11e3]  QLabcp=[100 90 110]  QCabcp=[100 90 110]  Measurements=None  LoadType=constant PQ
  Load23 : powerlib/Elements/Three-Phase Parallel RLC Load  LConnTagsString=A|B|C  Configuration=Y (grounded)  NominalVoltage=(278478)*1.00098  Vabc=[1e3 1e3 1e3]  Vabcp=[1e3 1e3 1e3]  NominalFrequency=50  UnbalancedPower=off  ActivePower=load_mag(23,2)*1e6  InductivePower=load_mag(23,3)*1e6  CapacitivePower=0  Pabc=[10e3 9e3 11e3]  QLabc=[100 90 110]  QCabc=[100 90 110]  Pabcp=[10e3 9e3 11e3]  QLabcp=[100 90 110]  QCabcp=[100 90 110]  Measurements=Branch voltages  LoadType=constant PQ
  Load24 : powerlib/Elements/Three-Phase Parallel RLC Load  LConnTagsString=A|B|C  Configuration=Y (grounded)  NominalVoltage=(275000)*1.01119  Vabc=[1e3 1e3 1e3]  Vabcp=[1e3 1e3 1e3]  NominalFrequency=50  UnbalancedPower=off  ActivePower=load_mag(24,2)*1e6  InductivePower=load_mag(24,3)*1e6  CapacitivePower=0  Pabc=[10e3 9e3 11e3]  QLabc=[100 90 110]  QCabc=[100 90 110]  Pabcp=[10e3 9e3 11e3]  QLabcp=[100 90 110]  QCabcp=[100 90 110]  Measurements=None  LoadType=constant PQ
  Load25 : powerlib/Elements/Three-Phase Parallel RLC Load  LConnTagsString=A|B|C  Configuration=Y (grounded)  NominalVoltage=(276329)*1.00111  Vabc=[1e3 1e3 1e3]  Vabcp=[1e3 1e3 1e3]  NominalFrequency=50  UnbalancedPower=off  ActivePower=load_mag(25,2)*1e6  InductivePower=load_mag(25,3)*1e6  CapacitivePower=0  Pabc=[10e3 9e3 11e3]  QLabc=[100 90 110]  QCabc=[100 90 110]  Pabcp=[10e3 9e3 11e3]  QLabcp=[100 90 110]  QCabcp=[100 90 110]  Measurements=None  LoadType=constant PQ
  Load26 : powerlib/Elements/Three-Phase Parallel RLC Load  LConnTagsString=A|B|C  Configuration=Y (grounded)  NominalVoltage=(285470)*1.00204  Vabc=[1e3 1e3 1e3]  Vabcp=[1e3 1e3 1e3]  NominalFrequency=50  UnbalancedPower=off  ActivePower=load_mag(26,2)*1e6  InductivePower=load_mag(26,3)*1e6  CapacitivePower=0  Pabc=[10e3 9e3 11e3]  QLabc=[100 90 110]  QCabc=[100 90 110]  Pabcp=[10e3 9e3 11e3]  QLabcp=[100 90 110]  QCabcp=[100 90 110]  Measurements=None  LoadType=constant PQ
  Load27 : powerlib/Elements/Three-Phase Parallel RLC Load  LConnTagsString=A|B|C  Configuration=Y (grounded)  NominalVoltage=(279067)*1.00215  Vabc=[1e3 1e3 1e3]  Vabcp=[1e3 1e3 1e3]  NominalFrequency=50  UnbalancedPower=off  ActivePower=load_mag(27,2)*1e6  InductivePower=load_mag(27,3)*1e6  CapacitivePower=0  Pabc=[10e3 9e3 11e3]  QLabc=[100 90 110]  QCabc=[100 90 110]  Pabcp=[10e3 9e3 11e3]  QLabcp=[100 90 110]  QCabcp=[100 90 110]  Measurements=None  LoadType=constant PQ
  Load28 : powerlib/Elements/Three-Phase Parallel RLC Load  LConnTagsString=A|B|C  Configuration=Y (grounded)  NominalVoltage=(277109)*1.00233  Vabc=[1e3 1e3 1e3]  Vabcp=[1e3 1e3 1e3]  NominalFrequency=50  UnbalancedPower=off  ActivePower=load_mag(28,2)*1e6  InductivePower=load_mag(28,3)*1e6  CapacitivePower=0  Pabc=[10e3 9e3 11e3]  QLabc=[100 90 110]  QCabc=[100 90 110]  Pabcp=[10e3 9e3 11e3]  QLabcp=[100 90 110]  QCabcp=[100 90 110]  Measurements=None  LoadType=constant PQ
  Load29 : powerlib/Elements/Three-Phase Parallel RLC Load  LConnTagsString=A|B|C  Configuration=Y (grounded)  NominalVoltage=(295429)*1.00282  Vabc=[1e3 1e3 1e3]  Vabcp=[1e3 1e3 1e3]  NominalFrequency=50  UnbalancedPower=off  ActivePower=load_mag(29,2)*1e6  InductivePower=load_mag(29,3)*1e6  CapacitivePower=0  Pabc=[10e3 9e3 11e3]  QLabc=[100 90 110]  QCabc=[100 90 110]  Pabcp=[10e3 9e3 11e3]  QLabcp=[100 90 110]  QCabcp=[100 90 110]  Measurements=None  LoadType=constant PQ
  Load3 : powerlib/Elements/Three-Phase Parallel RLC Load  LConnTagsString=A|B|C  Configuration=Y (grounded)  NominalVoltage=(335481)*1.00046  Vabc=[1e3 1e3 1e3]  Vabcp=[1e3 1e3 1e3]  NominalFrequency=50  UnbalancedPower=off  ActivePower=load_mag(3,2)*1e6  InductivePower=load_mag(3,3)*1e6  CapacitivePower=0  Pabc=[10e3 9e3 11e3]  QLabc=[100 90 110]  QCabc=[100 90 110]  Pabcp=[10e3 9e3 11e3]  QLabcp=[100 90 110]  QCabcp=[100 90 110]  Measurements=None  LoadType=constant PQ
  Load4 : powerlib/Elements/Three-Phase Parallel RLC Load  LConnTagsString=A|B|C  Configuration=Y (grounded)  NominalVoltage=(331947)*1.00076  Vabc=[1e3 1e3 1e3]  Vabcp=[1e3 1e3 1e3]  NominalFrequency=50  UnbalancedPower=off  ActivePower=load_mag(4,2)*1e6  InductivePower=load_mag(4,3)*1e6  CapacitivePower=0  Pabc=[10e3 9e3 11e3]  QLabc=[100 90 110]  QCabc=[100 90 110]  Pabcp=[10e3 9e3 11e3]  QLabcp=[100 90 110]  QCabcp=[100 90 110]  Measurements=None  LoadType=constant PQ
  Load5 : powerlib/Elements/Three-Phase Parallel RLC Load  LConnTagsString=A|B|C  Configuration=Y (grounded)  NominalVoltage=(332888)*1.00092  Vabc=[1e3 1e3 1e3]  Vabcp=[1e3 1e3 1e3]  NominalFrequency=50  UnbalancedPower=off  ActivePower=load_mag(5,2)*1e6  InductivePower=load_mag(5,3)*1e6  CapacitivePower=0  Pabc=[10e3 9e3 11e3]  QLabc=[100 90 110]  QCabc=[100 90 110]  Pabcp=[10e3 9e3 11e3]  QLabcp=[100 90 110]  QCabcp=[100 90 110]  Measurements=None  LoadType=constant PQ
  Load6 : powerlib/Elements/Three-Phase Parallel RLC Load  LConnTagsString=A|B|C  Configuration=Y (grounded)  NominalVoltage=(335217)*1.0013  Vabc=[1e3 1e3 1e3]  Vabcp=[1e3 1e3 1e3]  NominalFrequency=50  UnbalancedPower=off  ActivePower=load_mag(6,2)*1e6  InductivePower=load_mag(6,3)*1e6  CapacitivePower=0  Pabc=[10e3 9e3 11e3]  QLabc=[100 90 110]  QCabc=[100 90 110]  Pabcp=[10e3 9e3 11e3]  QLabcp=[100 90 110]  QCabcp=[100 90 110]  Measurements=None  LoadType=constant PQ
  Load7 : powerlib/Elements/Three-Phase Parallel RLC Load  LConnTagsString=A|B|C  Configuration=Y (grounded)  NominalVoltage=(330000)*1.02708  Vabc=[1e3 1e3 1e3]  Vabcp=[1e3 1e3 1e3]  NominalFrequency=50  UnbalancedPower=off  ActivePower=load_mag(7,2)*1e6  InductivePower=load_mag(7,3)*1e6  CapacitivePower=0  Pabc=[10e3 9e3 11e3]  QLabc=[100 90 110]  QCabc=[100 90 110]  Pabcp=[10e3 9e3 11e3]  QLabcp=[100 90 110]  QCabcp=[100 90 110]  Measurements=None  LoadType=constant PQ
  Load8 : powerlib/Elements/Three-Phase Parallel RLC Load  LConnTagsString=A|B|C  Configuration=Y (grounded)  NominalVoltage=(335416)*1.00085  Vabc=[1e3 1e3 1e3]  Vabcp=[1e3 1e3 1e3]  NominalFrequency=50  UnbalancedPower=off  ActivePower=load_mag(8,2)*1e6  InductivePower=load_mag(8,3)*1e6  CapacitivePower=0  Pabc=[10e3 9e3 11e3]  QLabc=[100 90 110]  QCabc=[100 90 110]  Pabcp=[10e3 9e3 11e3]  QLabcp=[100 90 110]  QCabcp=[100 90 110]  Measurements=None  LoadType=constant PQ
  Load9 : powerlib/Elements/Three-Phase Parallel RLC Load  LConnTagsString=A|B|C  Configuration=Y (grounded)  NominalVoltage=(330000)*1.03661  Vabc=[1e3 1e3 1e3]  Vabcp=[1e3 1e3 1e3]  NominalFrequency=50  UnbalancedPower=off  ActivePower=load_mag(9,2)*1e6  InductivePower=load_mag(9,3)*1e6  CapacitivePower=0  Pabc=[10e3 9e3 11e3]  QLabc=[100 90 110]  QCabc=[100 90 110]  Pabcp=[10e3 9e3 11e3]  QLabcp=[100 90 110]  QCabcp=[100 90 110]  Measurements=None  LoadType=constant PQ
  Measurements : Subsystem
  Mux{15..29} (15 alike) : Mux  Inputs=3
  P 1-3 : Scope  NumInputPorts=2
  P 2-1 : Scope  NumInputPorts=2
  P 3-5 : Scope  NumInputPorts=2
  P 4-2 : Scope  NumInputPorts=2
  PSS model : Constant  Value=PSSMODEL
  Scope : Scope
  Scope1 : Scope
  Scope4 : Scope  NumInputPorts=2
  T1 : powerlib/Elements/Three-Phase Transformer (Two Windings)  Winding1Connection=Yg  Winding2Connection=Yg  CoreType=Three single-phase transformers  SetSaturation=off  Hysteresis=off  DataFile='hysteresis'  SetInitialFlux=off  Measurements=None  UNITS=pu  NominalPower=[ trans(1,6)*1e6 , 50 ]  Winding1=[ trans(1,4)*1e3, 1e-6, 0 ]  Winding2=[ trans(1,5)*1e3, 1e-6, trans(1,7) ]  Rm=500  Lm=500  L0=0.5  Saturation=[ 0,0 ; 0.0024,1.2 ; 1.0,1.52 ]  InitialFluxes=[ 0.8 , -0.8 , 0.7 ]  MoreParameters=off  BreakLoop=off  DataType=off  TransfoNumber=0
  T10 : powerlib/Elements/Three-Phase Transformer (Two Windings)  Winding1Connection=Y  Winding2Connection=Y  CoreType=Three single-phase transformers  SetSaturation=off  Hysteresis=off  DataFile='hysteresis'  SetInitialFlux=off  Measurements=None  UNITS=pu  NominalPower=[ trans(10,6)*1e6 , 50 ]  Winding1=[ trans(10,4)*1e3, 1e-6 , 0 ]  Winding2=[ trans(10,5)*1e3, 0 , trans(10,7) ]  Rm=500  Lm=500  L0=0.5  Saturation=[ 0,0 ; 0.0024,1.2 ; 1.0,1.52 ]  InitialFluxes=[ 0.8 , -0.8 , 0.7 ]  MoreParameters=off  BreakLoop=off  DataType=off  TransfoNumber=0
  T11 : powerlib/Elements/Three-Phase Transformer (Two Windings)  Winding1Connection=Y  Winding2Connection=Y  CoreType=Three single-phase transformers  SetSaturation=off  Hysteresis=off  DataFile='hysteresis'  SetInitialFlux=off  Measurements=None  UNITS=pu  NominalPower=[ trans(11,6)*1e6 , 50 ]  Winding1=[ trans(11,4)*1e3, 1e-6, 0 ]  Winding2=[ trans(11,5)*1e3, 0 , trans(11,7) ]  Rm=500  Lm=500  L0=0.5  Saturation=[ 0,0 ; 0.0024,1.2 ; 1.0,1.52 ]  InitialFluxes=[ 0.8 , -0.8 , 0.7 ]  MoreParameters=off  BreakLoop=off  DataType=off  TransfoNumber=0
  T12 : powerlib/Elements/Three-Phase Transformer (Two Windings)  Winding1Connection=Y  Winding2Connection=Y  CoreType=Three single-phase transformers  SetSaturation=off  Hysteresis=off  DataFile='hysteresis'  SetInitialFlux=off  Measurements=None  UNITS=pu  NominalPower=[ trans(12,6)*1e6 , 50 ]  Winding1=[ trans(12,4)*1e3, 1e-6, 0 ]  Winding2=[ trans(12,5)*1e3, 0 , trans(12,7)]  Rm=500  Lm=500  L0=0.5  Saturation=[ 0,0 ; 0.0024,1.2 ; 1.0,1.52 ]  InitialFluxes=[ 0.8 , -0.8 , 0.7 ]  MoreParameters=off  BreakLoop=off  DataType=off  TransfoNumber=0
  T13 : powerlib/Elements/Three-Phase Transformer (Two Windings)  Winding1Connection=Y  Winding2Connection=Y  CoreType=Three single-phase transformers  SetSaturation=off  Hysteresis=off  DataFile='hysteresis'  SetInitialFlux=off  Measurements=None  UNITS=pu  NominalPower=[ trans(13,6)*1e6 , 50 ]  Winding1=[ trans(13,4)*1e3, 1e-6, 0 ]  Winding2=[ trans(13,5)*1e3, 0 , trans(13,7) ]  Rm=500  Lm=500  L0=0.5  Saturation=[ 0,0 ; 0.0024,1.2 ; 1.0,1.52 ]  InitialFluxes=[ 0.8 , -0.8 , 0.7 ]  MoreParameters=off  BreakLoop=off  DataType=off  TransfoNumber=0
  T14 : powerlib/Elements/Three-Phase Transformer (Two Windings)  Winding1Connection=Delta (D1)  Winding2Connection=Yg  CoreType=Three single-phase transformers  SetSaturation=off  Hysteresis=off  DataFile='hysteresis'  SetInitialFlux=off  Measurements=None  UNITS=pu  NominalPower=[ trans(14,6)*1e6 , 50 ]  Winding1=[ trans(14,4)*1e3, 1e-6 , 0 ]  Winding2=[ trans(14,5)*1e3, 0 , trans(14,7) ]  Rm=500  Lm=500  L0=0.5  Saturation=[ 0,0 ; 0.0024,1.2 ; 1.0,1.52 ]  InitialFluxes=[ 0.8 , -0.8 , 0.7 ]  MoreParameters=off  BreakLoop=off  DataType=off  TransfoNumber=0
  T15 : powerlib/Elements/Three-Phase Transformer (Two Windings)  Winding1Connection=Yg  Winding2Connection=Yg  CoreType=Three single-phase transformers  SetSaturation=off  Hysteresis=off  DataFile='hysteresis'  SetInitialFlux=off  Measurements=None  UNITS=pu  NominalPower=[ trans(15,6)*1e6 , 50 ]  Winding1=[ trans(15,4)*1e3, 1e-6 , 0 ]  Winding2=[ trans(15,5)*1e3, 0 , trans(15,7) ]  Rm=500  Lm=500  L0=0.5  Saturation=[ 0,0 ; 0.0024,1.2 ; 1.0,1.52 ]  InitialFluxes=[ 0.8 , -0.8 , 0.7 ]  MoreParameters=off  BreakLoop=off  DataType=off  TransfoNumber=0
  T16 : powerlib/Elements/Three-Phase Transformer (Two Windings)  Winding1Connection=Yg  Winding2Connection=Yg  CoreType=Three single-phase transformers  SetSaturation=off  Hysteresis=off  DataFile='hysteresis'  SetInitialFlux=off  Measurements=None  UNITS=pu  NominalPower=[ trans(16,6)*1e6 , 50 ]  Winding1=[ trans(16,4)*1e3, 1e-6 , 0]  Winding2=[ trans(16,5)*1e3, 0 , trans(16,7) ]  Rm=500  Lm=500  L0=0.5  Saturation=[ 0,0 ; 0.0024,1.2 ; 1.0,1.52 ]  InitialFluxes=[ 0.8 , -0.8 , 0.7 ]  MoreParameters=off  BreakLoop=off  DataType=off  TransfoNumber=0
  T17 : powerlib/Elements/Three-Phase Transformer (Two Windings)  Winding1Connection=Delta (D1)  Winding2Connection=Yg  CoreType=Three single-phase transformers  SetSaturation=off  Hysteresis=off  DataFile='hysteresis'  SetInitialFlux=off  Measurements=None  UNITS=pu  NominalPower=[ trans(17,6)*1e6 , 50 ]  Winding1=[ trans(17,4)*1e3, 1e-6 , 0 ]  Winding2=[ trans(17,5)*1e3, 0 , trans(17,7) ]  Rm=500  Lm=500  L0=0.5  Saturation=[ 0,0 ; 0.0024,1.2 ; 1.0,1.52 ]  InitialFluxes=[ 0.8 , -0.8 , 0.7 ]  MoreParameters=off  BreakLoop=off  DataType=off  TransfoNumber=0
  T18 : powerlib/Elements/Three-Phase Transformer (Two Windings)  Winding1Connection=Yg  Winding2Connection=Yg  CoreType=Three single-phase transformers  SetSaturation=off  Hysteresis=off  DataFile='hysteresis'  SetInitialFlux=off  Measurements=None  UNITS=pu  NominalPower=[ trans(9,6)*1e6 , 50 ]  Winding1=[ trans(9,4)*1e3, 1e-6, 0 ]  Winding2=[ trans(9,5)*1e3, 0 , trans(9,7)]  Rm=500  Lm=500  L0=0.5  Saturation=[ 0,0 ; 0.0024,1.2 ; 1.0,1.52 ]  InitialFluxes=[ 0.8 , -0.8 , 0.7 ]  MoreParameters=off  BreakLoop=off  DataType=off  TransfoNumber=0
  T18-1 : powerlib/Elements/Three-Phase Transformer (Two Windings)  Winding1Connection=Y  Winding2Connection=Y  CoreType=Three single-phase transformers  SetSaturation=off  Hysteresis=off  DataFile='hysteresis'  SetInitialFlux=off  Measurements=None  UNITS=pu  NominalPower=[ trans(18,6)*1e6 , 50 ]  Winding1=[ trans(18,4)*1e3, 1e-6, 0 ]  Winding2=[ trans(18,5)*1e3, 0 , trans(18,7) ]  Rm=500  Lm=500  L0=0.5  Saturation=[ 0,0 ; 0.0024,1.2 ; 1.0,1.52 ]  InitialFluxes=[ 0.8 , -0.8 , 0.7 ]  MoreParameters=off  BreakLoop=off  DataType=off  TransfoNumber=0
  T18-2 : powerlib/Elements/Three-Phase Transformer (Two Windings)  Winding1Connection=Y  Winding2Connection=Y  CoreType=Three single-phase transformers  SetSaturation=off  Hysteresis=off  DataFile='hysteresis'  SetInitialFlux=off  Measurements=None  UNITS=pu  NominalPower=[ trans(18,6)*1e6 , 50 ]  Winding1=[ trans(18,4)*1e3, 1e-6, 0 ]  Winding2=[ trans(18,5)*1e3, 0 , trans(18,7) ]  Rm=500  Lm=500  L0=0.5  Saturation=[ 0,0 ; 0.0024,1.2 ; 1.0,1.52 ]  InitialFluxes=[ 0.8 , -0.8 , 0.7 ]  MoreParameters=off  BreakLoop=off  DataType=off  TransfoNumber=0
  T19 : powerlib/Elements/Three-Phase Transformer (Two Windings)  Winding1Connection=Delta (D1)  Winding2Connection=Yg  CoreType=Three single-phase transformers  SetSaturation=off  Hysteresis=off  DataFile='hysteresis'  SetInitialFlux=off  Measurements=None  UNITS=pu  NominalPower=[ trans(19,6)*1e6 , 50 ]  Winding1=[ trans(19,4)*1e3, 1e-6 , 0 ]  Winding2=[ trans(19,5)*1e3, 0 , trans(19,7) ]  Rm=500  Lm=500  L0=0.5  Saturation=[ 0,0 ; 0.0024,1.2 ; 1.0,1.52 ]  InitialFluxes=[ 0.8 , -0.8 , 0.7 ]  MoreParameters=off  BreakLoop=off  DataType=off  TransfoNumber=0
  T2 : powerlib/Elements/Three-Phase Transformer (Two Windings)  Winding1Connection=Delta (D1)  Winding2Connection=Yg  CoreType=Three single-phase transformers  SetSaturation=off  Hysteresis=off  DataFile='hysteresis'  SetInitialFlux=off  Measurements=None  UNITS=pu  NominalPower=[ trans(2,6)*1e6 , 50 ]  Winding1=[ trans(2,4)*1e3, 1e-6 , 0 ]  Winding2=[ trans(2,5)*1e3, 0 , trans(2,7) ]  Rm=500  Lm=500  L0=0.5  Saturation=[ 0,0 ; 0.0024,1.2 ; 1.0,1.52 ]  InitialFluxes=[ 0.8 , -0.8 , 0.7 ]  MoreParameters=off  BreakLoop=off  DataType=off  TransfoNumber=0
  T20 : powerlib/Elements/Three-Phase Transformer (Two Windings)  Winding1Connection=Yg  Winding2Connection=Yg  CoreType=Three single-phase transformers  SetSaturation=off  Hysteresis=off  DataFile='hysteresis'  SetInitialFlux=off  Measurements=None  UNITS=pu  NominalPower=[ trans(20,6)*1e6 , 50 ]  Winding1=[ trans(20,4)*1e3, 1e-6 , 0]  Winding2=[ trans(20,5)*1e3, 0 , trans(20,7) ]  Rm=500  Lm=500  L0=0.5  Saturation=[ 0,0 ; 0.0024,1.2 ; 1.0,1.52 ]  InitialFluxes=[ 0.8 , -0.8 , 0.7 ]  MoreParameters=off  BreakLoop=off  DataType=off  TransfoNumber=0
  T21 : powerlib/Elements/Three-Phase Transformer (Two Windings)  Winding1Connection=Delta (D1)  Winding2Connection=Yg  CoreType=Three single-phase transformers  SetSaturation=off  Hysteresis=off  DataFile='hysteresis'  SetInitialFlux=off  Measurements=None  UNITS=pu  NominalPower=[ trans(21,6)*1e6 , 50 ]  Winding1=[ trans(21,4)*1e3, 1e-6 , 0 ]  Winding2=[ trans(21,5)*1e3, 0 , trans(21,7) ]  Rm=500  Lm=500  L0=0.5  Saturation=[ 0,0 ; 0.0024,1.2 ; 1.0,1.52 ]  InitialFluxes=[ 0.8 , -0.8 , 0.7 ]  MoreParameters=off  BreakLoop=off  DataType=off  TransfoNumber=0
  T22 : powerlib/Elements/Three-Phase Transformer (Two Windings)  Winding1Connection=Yg  Winding2Connection=Yg  CoreType=Three single-phase transformers  SetSaturation=off  Hysteresis=off  DataFile='hysteresis'  SetInitialFlux=off  Measurements=None  UNITS=pu  NominalPower=[ trans(9,6)*1e6 , 50 ]  Winding1=[ trans(9,4)*1e3, 1e-6, 0 ]  Winding2=[ trans(9,5)*1e3, 0 , trans(9,7)]  Rm=500  Lm=500  L0=0.5  Saturation=[ 0,0 ; 0.0024,1.2 ; 1.0,1.52 ]  InitialFluxes=[ 0.8 , -0.8 , 0.7 ]  MoreParameters=off  BreakLoop=off  DataType=off  TransfoNumber=0
  T23 : powerlib/Elements/Three-Phase Transformer (Two Windings)  Winding1Connection=Yg  Winding2Connection=Yg  CoreType=Three single-phase transformers  SetSaturation=off  Hysteresis=off  DataFile='hysteresis'  SetInitialFlux=off  Measurements=None  UNITS=pu  NominalPower=[ trans(8,6)*1e6 , 50 ]  Winding1=[ trans(8,4)*1e3, 1e-6 , 0 ]  Winding2=[ trans(8,5)*1e3, 0 , trans(8,7)]  Rm=500  Lm=500  L0=0.5  Saturation=[ 0,0 ; 0.0024,1.2 ; 1.0,1.52 ]  InitialFluxes=[ 0.8 , -0.8 , 0.7 ]  MoreParameters=off  BreakLoop=off  DataType=off  TransfoNumber=0
  T24 : powerlib/Elements/Three-Phase Transformer (Two Windings)  Winding1Connection=Yg  Winding2Connection=Yg  CoreType=Three single-phase transformers  SetSaturation=off  Hysteresis=off  DataFile='hysteresis'  SetInitialFlux=off  Measurements=None  UNITS=pu  NominalPower=[ trans(21,6)*1e6 , 50 ]  Winding1=[ trans(21,4)*1e3, 1e-6 , 0 ]  Winding2=[ trans(21,5)*1e3, 0 , trans(21,7) ]  Rm=500  Lm=500  L0=0.5  Saturation=[ 0,0 ; 0.0024,1.2 ; 1.0,1.52 ]  InitialFluxes=[ 0.8 , -0.8 , 0.7 ]  MoreParameters=off  BreakLoop=off  DataType=off  TransfoNumber=0
  T25 : powerlib/Elements/Three-Phase Transformer (Two Windings)  Winding1Connection=Yg  Winding2Connection=Yg  CoreType=Three single-phase transformers  SetSaturation=off  Hysteresis=off  DataFile='hysteresis'  SetInitialFlux=off  Measurements=None  UNITS=pu  NominalPower=[ trans(19,6)*1e6 , 50 ]  Winding1=[ trans(19,4)*1e3, 1e-6 , 0 ]  Winding2=[ trans(19,5)*1e3, 0 , trans(19,7) ]  Rm=500  Lm=500  L0=0.5  Saturation=[ 0,0 ; 0.0024,1.2 ; 1.0,1.52 ]  InitialFluxes=[ 0.8 , -0.8 , 0.7 ]  MoreParameters=off  BreakLoop=off  DataType=off  TransfoNumber=0
  T26 : powerlib/Elements/Three-Phase Transformer (Two Windings)  Winding1Connection=Yg  Winding2Connection=Yg  CoreType=Three single-phase transformers  SetSaturation=off  Hysteresis=off  DataFile='hysteresis'  SetInitialFlux=off  Measurements=None  UNITS=pu  NominalPower=[ trans(1,6)*1e6 , 50 ]  Winding1=[ trans(1,4)*1e3, 1e-6, 0 ]  Winding2=[ trans(1,5)*1e3, 1e-6, trans(1,7) ]  Rm=500  Lm=500  L0=0.5  Saturation=[ 0,0 ; 0.0024,1.2 ; 1.0,1.52 ]  InitialFluxes=[ 0.8 , -0.8 , 0.7 ]  MoreParameters=off  BreakLoop=off  DataType=off  TransfoNumber=0
  T27 : powerlib/Elements/Three-Phase Transformer (Two Windings)  Winding1Connection=Yg  Winding2Connection=Yg  CoreType=Three single-phase transformers  SetSaturation=off  Hysteresis=off  DataFile='hysteresis'  SetInitialFlux=off  Measurements=None  UNITS=pu  NominalPower=[ trans(1,6)*1e6 , 50 ]  Winding1=[ trans(1,4)*1e3, 1e-6, 0 ]  Winding2=[ trans(1,5)*1e3, 1e-6, trans(1,7) ]  Rm=500  Lm=500  L0=0.5  Saturation=[ 0,0 ; 0.0024,1.2 ; 1.0,1.52 ]  InitialFluxes=[ 0.8 , -0.8 , 0.7 ]  MoreParameters=off  BreakLoop=off  DataType=off  TransfoNumber=0
  T28 : powerlib/Elements/Three-Phase Transformer (Two Windings)  Winding1Connection=Yg  Winding2Connection=Yg  CoreType=Three single-phase transformers  SetSaturation=off  Hysteresis=off  DataFile='hysteresis'  SetInitialFlux=off  Measurements=None  UNITS=pu  NominalPower=[ trans(4,6)*1e6 , 50 ]  Winding1=[ trans(4,4)*1e3, 1e-6 , 0 ]  Winding2=[ trans(4,5)*1e3, 0 , trans(4,7) ]  Rm=500  Lm=500  L0=0.5  Saturation=[ 0,0 ; 0.0024,1.2 ; 1.0,1.52 ]  InitialFluxes=[ 0.8 , -0.8 , 0.7 ]  MoreParameters=off  BreakLoop=off  DataType=off  TransfoNumber=0
  T29 : powerlib/Elements/Three-Phase Transformer (Two Windings)  Winding1Connection=Yg  Winding2Connection=Yg  CoreType=Three single-phase transformers  SetSaturation=off  Hysteresis=off  DataFile='hysteresis'  SetInitialFlux=off  Measurements=None  UNITS=pu  NominalPower=[ trans(5,6)*1e6 , 50 ]  Winding1=[ trans(5,4)*1e3, 1e-6 , 0 ]  Winding2=[ trans(5,5)*1e3, 0 , trans(5,7) ]  Rm=500  Lm=500  L0=0.5  Saturation=[ 0,0 ; 0.0024,1.2 ; 1.0,1.52 ]  InitialFluxes=[ 0.8 , -0.8 , 0.7 ]  MoreParameters=off  BreakLoop=off  DataType=off  TransfoNumber=0
  T3 : powerlib/Elements/Three-Phase Transformer (Two Windings)  Winding1Connection=Delta (D1)  Winding2Connection=Yg  CoreType=Three single-phase transformers  SetSaturation=off  Hysteresis=off  DataFile='hysteresis'  SetInitialFlux=off  Measurements=None  UNITS=pu  NominalPower=[ trans(3,6)*1e6 , 50 ]  Winding1=[ trans(3,4)*1e3, 1e-6 , 0 ]  Winding2=[ trans(3,5)*1e3, 0 , trans(3,7) ]  Rm=500  Lm=500  L0=0.5  Saturation=[ 0,0 ; 0.0024,1.2 ; 1.0,1.52 ]  InitialFluxes=[ 0.8 , -0.8 , 0.7 ]  MoreParameters=off  BreakLoop=off  DataType=off  TransfoNumber=0
  T30 : powerlib/Elements/Three-Phase Transformer (Two Windings)  Winding1Connection=Yg  Winding2Connection=Yg  CoreType=Three single-phase transformers  SetSaturation=off  Hysteresis=off  DataFile='hysteresis'  SetInitialFlux=off  Measurements=None  UNITS=pu  NominalPower=[ trans(5,6)*1e6 , 50 ]  Winding1=[ trans(5,4)*1e3, 1e-6 , 0 ]  Winding2=[ trans(5,5)*1e3, 0 , trans(5,7) ]  Rm=500  Lm=500  L0=0.5  Saturation=[ 0,0 ; 0.0024,1.2 ; 1.0,1.52 ]  InitialFluxes=[ 0.8 , -0.8 , 0.7 ]  MoreParameters=off  BreakLoop=off  DataType=off  TransfoNumber=0
  T31 : powerlib/Elements/Three-Phase Transformer (Two Windings)  Winding1Connection=Yg  Winding2Connection=Yg  CoreType=Three single-phase transformers  SetSaturation=off  Hysteresis=off  DataFile='hysteresis'  SetInitialFlux=off  Measurements=None  UNITS=pu  NominalPower=[ trans(4,6)*1e6 , 50 ]  Winding1=[ trans(4,4)*1e3, 1e-6 , 0 ]  Winding2=[ trans(4,5)*1e3, 0 , trans(4,7) ]  Rm=500  Lm=500  L0=0.5  Saturation=[ 0,0 ; 0.0024,1.2 ; 1.0,1.52 ]  InitialFluxes=[ 0.8 , -0.8 , 0.7 ]  MoreParameters=off  BreakLoop=off  DataType=off  TransfoNumber=0
  T32 : powerlib/Elements/Three-Phase Transformer (Two Windings)  Winding1Connection=Yg  Winding2Connection=Yg  CoreType=Three single-phase transformers  SetSaturation=off  Hysteresis=off  DataFile='hysteresis'  SetInitialFlux=off  Measurements=None  UNITS=pu  NominalPower=[ trans(14,6)*1e6 , 50 ]  Winding1=[ trans(14,4)*1e3, 1e-6 , 0 ]  Winding2=[ trans(14,5)*1e3, 0 , trans(14,7) ]  Rm=500  Lm=500  L0=0.5  Saturation=[ 0,0 ; 0.0024,1.2 ; 1.0,1.52 ]  InitialFluxes=[ 0.8 , -0.8 , 0.7 ]  MoreParameters=off  BreakLoop=off  DataType=off  TransfoNumber=0
  T33 : powerlib/Elements/Three-Phase Transformer (Two Windings)  Winding1Connection=Yg  Winding2Connection=Yg  CoreType=Three single-phase transformers  SetSaturation=off  Hysteresis=off  DataFile='hysteresis'  SetInitialFlux=off  Measurements=None  UNITS=pu  NominalPower=[ trans(17,6)*1e6 , 50 ]  Winding1=[ trans(17,4)*1e3, 1e-6 , 0 ]  Winding2=[ trans(17,5)*1e3, 0 , trans(17,7) ]  Rm=500  Lm=500  L0=0.5  Saturation=[ 0,0 ; 0.0024,1.2 ; 1.0,1.52 ]  InitialFluxes=[ 0.8 , -0.8 , 0.7 ]  MoreParameters=off  BreakLoop=off  DataType=off  TransfoNumber=0
  T34 : powerlib/Elements/Three-Phase Transformer (Two Windings)  Winding1Connection=Yg  Winding2Connection=Yg  CoreType=Three single-phase transformers  SetSaturation=off  Hysteresis=off  DataFile='hysteresis'  SetInitialFlux=off  Measurements=None  UNITS=pu  NominalPower=[ trans(19,6)*1e6 , 50 ]  Winding1=[ trans(19,4)*1e3, 1e-6 , 0 ]  Winding2=[ trans(19,5)*1e3, 0 , trans(19,7) ]  Rm=500  Lm=500  L0=0.5  Saturation=[ 0,0 ; 0.0024,1.2 ; 1.0,1.52 ]  InitialFluxes=[ 0.8 , -0.8 , 0.7 ]  MoreParameters=off  BreakLoop=off  DataType=off  TransfoNumber=0
  T35 : powerlib/Elements/Three-Phase Transformer (Two Windings)  Winding1Connection=Yg  Winding2Connection=Yg  CoreType=Three single-phase transformers  SetSaturation=off  Hysteresis=off  DataFile='hysteresis'  SetInitialFlux=off  Measurements=None  UNITS=pu  NominalPower=[ trans(14,6)*1e6 , 50 ]  Winding1=[ trans(14,4)*1e3, 1e-6 , 0 ]  Winding2=[ trans(14,5)*1e3, 0 , trans(14,7) ]  Rm=500  Lm=500  L0=0.5  Saturation=[ 0,0 ; 0.0024,1.2 ; 1.0,1.52 ]  InitialFluxes=[ 0.8 , -0.8 , 0.7 ]  MoreParameters=off  BreakLoop=off  DataType=off  TransfoNumber=0
  T36 : powerlib/Elements/Three-Phase Transformer (Two Windings)  Winding1Connection=Yg  Winding2Connection=Yg  CoreType=Three single-phase transformers  SetSaturation=off  Hysteresis=off  DataFile='hysteresis'  SetInitialFlux=off  Measurements=None  UNITS=pu  NominalPower=[ trans(14,6)*1e6 , 50 ]  Winding1=[ trans(14,4)*1e3, 1e-6 , 0 ]  Winding2=[ trans(14,5)*1e3, 0 , trans(14,7) ]  Rm=500  Lm=500  L0=0.5  Saturation=[ 0,0 ; 0.0024,1.2 ; 1.0,1.52 ]  InitialFluxes=[ 0.8 , -0.8 , 0.7 ]  MoreParameters=off  BreakLoop=off  DataType=off  TransfoNumber=0
  T37 : powerlib/Elements/Three-Phase Transformer (Two Windings)  Winding1Connection=Yg  Winding2Connection=Yg  CoreType=Three single-phase transformers  SetSaturation=off  Hysteresis=off  DataFile='hysteresis'  SetInitialFlux=off  Measurements=None  UNITS=pu  NominalPower=[ trans(2,6)*1e6 , 50 ]  Winding1=[ trans(2,4)*1e3, 1e-6 , 0 ]  Winding2=[ trans(2,5)*1e3, 0 , trans(2,7) ]  Rm=500  Lm=500  L0=0.5  Saturation=[ 0,0 ; 0.0024,1.2 ; 1.0,1.52 ]  InitialFluxes=[ 0.8 , -0.8 , 0.7 ]  MoreParameters=off  BreakLoop=off  DataType=off  TransfoNumber=0
  T38 : powerlib/Elements/Three-Phase Transformer (Two Windings)  Winding1Connection=Yg  Winding2Connection=Yg  CoreType=Three single-phase transformers  SetSaturation=off  Hysteresis=off  DataFile='hysteresis'  SetInitialFlux=off  Measurements=None  UNITS=pu  NominalPower=[ trans(4,6)*1e6 , 50 ]  Winding1=[ trans(4,4)*1e3, 1e-6 , 0 ]  Winding2=[ trans(4,5)*1e3, 0 , trans(4,7) ]  Rm=500  Lm=500  L0=0.5  Saturation=[ 0,0 ; 0.0024,1.2 ; 1.0,1.52 ]  InitialFluxes=[ 0.8 , -0.8 , 0.7 ]  MoreParameters=off  BreakLoop=off  DataType=off  TransfoNumber=0
  T39 : powerlib/Elements/Three-Phase Transformer (Two Windings)  Winding1Connection=Yg  Winding2Connection=Yg  CoreType=Three single-phase transformers  SetSaturation=off  Hysteresis=off  DataFile='hysteresis'  SetInitialFlux=off  Measurements=None  UNITS=pu  NominalPower=[ trans(8,6)*1e6 , 50 ]  Winding1=[ trans(8,4)*1e3, 1e-6 , 0 ]  Winding2=[ trans(8,5)*1e3, 0 , trans(8,7)]  Rm=500  Lm=500  L0=0.5  Saturation=[ 0,0 ; 0.0024,1.2 ; 1.0,1.52 ]  InitialFluxes=[ 0.8 , -0.8 , 0.7 ]  MoreParameters=off  BreakLoop=off  DataType=off  TransfoNumber=0
  T4 : powerlib/Elements/Three-Phase Transformer (Two Windings)  Winding1Connection=Delta (D1)  Winding2Connection=Yg  CoreType=Three single-phase transformers  SetSaturation=off  Hysteresis=off  DataFile='hysteresis'  SetInitialFlux=off  Measurements=None  UNITS=pu  NominalPower=[ trans(4,6)*1e6 , 50 ]  Winding1=[ trans(4,4)*1e3, 1e-6 , 0 ]  Winding2=[ trans(4,5)*1e3, 0 , trans(4,7) ]  Rm=500  Lm=500  L0=0.5  Saturation=[ 0,0 ; 0.0024,1.2 ; 1.0,1.52 ]  InitialFluxes=[ 0.8 , -0.8 , 0.7 ]  MoreParameters=off  BreakLoop=off  DataType=off  TransfoNumber=0
  T40 : powerlib/Elements/Three-Phase Transformer (Two Windings)  Winding1Connection=Yg  Winding2Connection=Yg  CoreType=Three single-phase transformers  SetSaturation=off  Hysteresis=off  DataFile='hysteresis'  SetInitialFlux=off  Measurements=None  UNITS=pu  NominalPower=[ trans(21,6)*1e6 , 50 ]  Winding1=[ trans(21,4)*1e3, 1e-6 , 0 ]  Winding2=[ trans(21,5)*1e3, 0 , trans(21,7) ]  Rm=500  Lm=500  L0=0.5  Saturation=[ 0,0 ; 0.0024,1.2 ; 1.0,1.52 ]  InitialFluxes=[ 0.8 , -0.8 , 0.7 ]  MoreParameters=off  BreakLoop=off  DataType=off  TransfoNumber=0
  T5 : powerlib/Elements/Three-Phase Transformer (Two Windings)  Winding1Connection=Delta (D1)  Winding2Connection=Yg  CoreType=Three single-phase transformers  SetSaturation=off  Hysteresis=off  DataFile='hysteresis'  SetInitialFlux=off  Measurements=None  UNITS=pu  NominalPower=[ trans(5,6)*1e6 , 50 ]  Winding1=[ trans(5,4)*1e3, 1e-6 , 0 ]  Winding2=[ trans(5,5)*1e3, 0 , trans(5,7) ]  Rm=500  Lm=500  L0=0.5  Saturation=[ 0,0 ; 0.0024,1.2 ; 1.0,1.52 ]  InitialFluxes=[ 0.8 , -0.8 , 0.7 ]  MoreParameters=off  BreakLoop=off  DataType=off  TransfoNumber=0
  T6 : powerlib/Elements/Three-Phase Transformer (Two Windings)  Winding1Connection=Y  Winding2Connection=Y  CoreType=Three single-phase transformers  SetSaturation=off  Hysteresis=off  DataFile='hysteresis'  SetInitialFlux=off  Measurements=None  UNITS=pu  NominalPower=[ trans(6,6)*1e6 , 50 ]  Winding1="[ trans(6,4)*1e3, 1e-6, 0  ]"  Winding2=[ trans(6,5)*1e3, 0 , trans(6,7)]  Rm=500  Lm=500  L0=0.5  Saturation=[ 0,0 ; 0.0024,1.2 ; 1.0,1.52 ]  InitialFluxes=[ 0.8 , -0.8 , 0.7 ]  MoreParameters=off  BreakLoop=off  DataType=off  TransfoNumber=0
  T7 : powerlib/Elements/Three-Phase Transformer (Two Windings)  Winding1Connection=Y  Winding2Connection=Y  CoreType=Three single-phase transformers  SetSaturation=off  Hysteresis=off  DataFile='hysteresis'  SetInitialFlux=off  Measurements=None  UNITS=pu  NominalPower=[ trans(7,6)*1e6 , 50 ]  Winding1=[ trans(7,4)*1e3, 1e-6, 0 ]  Winding2=[ trans(7,5)*1e3, 0 , trans(7,7) ]  Rm=500  Lm=500  L0=0.5  Saturation=[ 0,0 ; 0.0024,1.2 ; 1.0,1.52 ]  InitialFluxes=[ 0.8 , -0.8 , 0.7 ]  MoreParameters=off  BreakLoop=off  DataType=off  TransfoNumber=0
  T8 : powerlib/Elements/Three-Phase Transformer (Two Windings)  Winding1Connection=Delta (D1)  Winding2Connection=Yg  CoreType=Three single-phase transformers  SetSaturation=off  Hysteresis=off  DataFile='hysteresis'  SetInitialFlux=off  Measurements=None  UNITS=pu  NominalPower=[ trans(8,6)*1e6 , 50 ]  Winding1=[ trans(8,4)*1e3, 1e-6 , 0 ]  Winding2=[ trans(8,5)*1e3, 0 , trans(8,7)]  Rm=500  Lm=500  L0=0.5  Saturation=[ 0,0 ; 0.0024,1.2 ; 1.0,1.52 ]  InitialFluxes=[ 0.8 , -0.8 , 0.7 ]  MoreParameters=off  BreakLoop=off  DataType=off  TransfoNumber=0
  T9 : powerlib/Elements/Three-Phase Transformer (Two Windings)  Winding1Connection=Delta (D1)  Winding2Connection=Yg  CoreType=Three single-phase transformers  SetSaturation=off  Hysteresis=off  DataFile='hysteresis'  SetInitialFlux=off  Measurements=None  UNITS=pu  NominalPower=[ trans(9,6)*1e6 , 50 ]  Winding1=[ trans(9,4)*1e3, 1e-6, 0 ]  Winding2=[ trans(9,5)*1e3, 0 , trans(9,7)]  Rm=500  Lm=500  L0=0.5  Saturation=[ 0,0 ; 0.0024,1.2 ; 1.0,1.52 ]  InitialFluxes=[ 0.8 , -0.8 , 0.7 ]  MoreParameters=off  BreakLoop=off  DataType=off  TransfoNumber=0
  Three-Phase V-I Measurement{1..5} (5 alike) : powerlib/Measurements/Three-Phase V-I Measurement  VoltageMeasurement=phase-to-ground  SetLabelV=off  LabelV=Vabc  Vpu=off  VpuLL=off  CurrentMeasurement=yes  SetLabelI=off  LabelI=Iabc  Ipu=off  Pbase=100e6  Vbase=500e3  OutputType=Complex  PhasorSimulation=on  PSBequivalent=0
  Voltage Measurement : powerlib/Measurements/Voltage Measurement  PhasorSimulation=on  OutputType=Magnitude  PSBequivalent=0
  fake_VSC_2 : powerlib/Electrical Sources/Three-Phase Source  Commented=on  InternalConnection=Yg  VoltagePhases=off  Voltage=(15000)*1  PhaseAngle=6.6166  Voltage_phases=[25e3 25e3 25e3]/sqrt(3)  PhaseAngles_phases=[0 -120 +120]  Frequency=50  NonIdealSource=off  SpecifyImpedance=off  Resistance=0  Inductance=0  ShortCircuitLevel=100e6  BaseVoltage=20e3  XRratio=7  BusType=PV  Pref=0  Qref=0  Prefabc=[10e3, 10e3, 10e3]  Qrefabc=[0, 0, 0]  Qmin=-inf  Qmax=inf
  fake_VSC_208 : powerlib/Electrical Sources/Three-Phase Source  Commented=on  InternalConnection=Yg  VoltagePhases=off  Voltage=(20000)*1  PhaseAngle=21.2703  Voltage_phases=[25e3 25e3 25e3]/sqrt(3)  PhaseAngles_phases=[0 -120 +120]  Frequency=50  NonIdealSource=off  SpecifyImpedance=off  Resistance=0  Inductance=0  ShortCircuitLevel=100e6  BaseVoltage=20e3  XRratio=7  BusType=PV  Pref=0  Qref=0  Prefabc=[10e3, 10e3, 10e3]  Qrefabc=[0, 0, 0]  Qmin=-inf  Qmax=inf
  fake_VSC_212 : powerlib/Electrical Sources/Three-Phase Source  Commented=on  InternalConnection=Yg  VoltagePhases=off  Voltage=(20000)*1  PhaseAngle=15.5222  Voltage_phases=[25e3 25e3 25e3]/sqrt(3)  PhaseAngles_phases=[0 -120 +120]  Frequency=50  NonIdealSource=off  SpecifyImpedance=off  Resistance=0  Inductance=0  ShortCircuitLevel=100e6  BaseVoltage=20e3  XRratio=7  BusType=PV  Pref=0  Qref=0  Prefabc=[10e3, 10e3, 10e3]  Qrefabc=[0, 0, 0]  Qmin=-inf  Qmax=inf
  fake_VSC_215 : powerlib/Electrical Sources/Three-Phase Source  Commented=on  InternalConnection=Yg  VoltagePhases=off  Voltage=(20000)*1  PhaseAngle=23.8703  Voltage_phases=[25e3 25e3 25e3]/sqrt(3)  PhaseAngles_phases=[0 -120 +120]  Frequency=50  NonIdealSource=off  SpecifyImpedance=off  Resistance=0  Inductance=0  ShortCircuitLevel=100e6  BaseVoltage=20e3  XRratio=7  BusType=PV  Pref=0  Qref=0  Prefabc=[10e3, 10e3, 10e3]  Qrefabc=[0, 0, 0]  Qmin=-inf  Qmax=inf
  fake_VSC_216 : powerlib/Electrical Sources/Three-Phase Source  Commented=on  InternalConnection=Yg  VoltagePhases=off  Voltage=(20000)*1  PhaseAngle=14.0249  Voltage_phases=[25e3 25e3 25e3]/sqrt(3)  PhaseAngles_phases=[0 -120 +120]  Frequency=50  NonIdealSource=off  SpecifyImpedance=off  Resistance=0  Inductance=0  ShortCircuitLevel=100e6  BaseVoltage=20e3  XRratio=7  BusType=PV  Pref=0  Qref=0  Prefabc=[10e3, 10e3, 10e3]  Qrefabc=[0, 0, 0]  Qmin=-inf  Qmax=inf
  fake_VSC_308 : powerlib/Electrical Sources/Three-Phase Source  Commented=on  InternalConnection=Yg  VoltagePhases=off  Voltage=(20000)*1  PhaseAngle=-6.3379  Voltage_phases=[25e3 25e3 25e3]/sqrt(3)  PhaseAngles_phases=[0 -120 +120]  Frequency=50  NonIdealSource=off  SpecifyImpedance=off  Resistance=0  Inductance=0  ShortCircuitLevel=100e6  BaseVoltage=20e3  XRratio=7  BusType=PV  Pref=0  Qref=0  Prefabc=[10e3, 10e3, 10e3]  Qrefabc=[0, 0, 0]  Qmin=-inf  Qmax=inf
  fake_VSC_309 : powerlib/Electrical Sources/Three-Phase Source  Commented=on  InternalConnection=Yg  VoltagePhases=off  Voltage=(15000)*1  PhaseAngle=4.7928  Voltage_phases=[25e3 25e3 25e3]/sqrt(3)  PhaseAngles_phases=[0 -120 +120]  Frequency=50  NonIdealSource=off  SpecifyImpedance=off  Resistance=0  Inductance=0  ShortCircuitLevel=100e6  BaseVoltage=20e3  XRratio=7  BusType=PV  Pref=0  Qref=0  Prefabc=[10e3, 10e3, 10e3]  Qrefabc=[0, 0, 0]  Qmin=-inf  Qmax=inf
  fake_VSC_312 : powerlib/Electrical Sources/Three-Phase Source  Commented=on  InternalConnection=Yg  VoltagePhases=off  Voltage=(20000)*1  PhaseAngle=3.6837  Voltage_phases=[25e3 25e3 25e3]/sqrt(3)  PhaseAngles_phases=[0 -120 +120]  Frequency=50  NonIdealSource=off  SpecifyImpedance=off  Resistance=0  Inductance=0  ShortCircuitLevel=100e6  BaseVoltage=20e3  XRratio=7  BusType=PV  Pref=0  Qref=0  Prefabc=[10e3, 10e3, 10e3]  Qrefabc=[0, 0, 0]  Qmin=-inf  Qmax=inf
  fake_VSC_314 : powerlib/Electrical Sources/Three-Phase Source  Commented=on  InternalConnection=Yg  VoltagePhases=off  Voltage=(20000)*1  PhaseAngle=-1.0986  Voltage_phases=[25e3 25e3 25e3]/sqrt(3)  PhaseAngles_phases=[0 -120 +120]  Frequency=50  NonIdealSource=off  SpecifyImpedance=off  Resistance=0  Inductance=0  ShortCircuitLevel=100e6  BaseVoltage=20e3  XRratio=7  BusType=PV  Pref=0  Qref=0  Prefabc=[10e3, 10e3, 10e3]  Qrefabc=[0, 0, 0]  Qmin=-inf  Qmax=inf
  fake_VSC_403 : powerlib/Electrical Sources/Three-Phase Source  Commented=on  InternalConnection=Yg  VoltagePhases=off  Voltage=(20000)*1  PhaseAngle=23.5812  Voltage_phases=[25e3 25e3 25e3]/sqrt(3)  PhaseAngles_phases=[0 -120 +120]  Frequency=50  NonIdealSource=off  SpecifyImpedance=off  Resistance=0  Inductance=0  ShortCircuitLevel=100e6  BaseVoltage=20e3  XRratio=7  BusType=PV  Pref=0  Qref=0  Prefabc=[10e3, 10e3, 10e3]  Qrefabc=[0, 0, 0]  Qmin=-inf  Qmax=inf
  fake_VSC_405 : powerlib/Electrical Sources/Three-Phase Source  Commented=on  InternalConnection=Yg  VoltagePhases=off  Voltage=(20000)*1  PhaseAngle=10.5944  Voltage_phases=[25e3 25e3 25e3]/sqrt(3)  PhaseAngles_phases=[0 -120 +120]  Frequency=50  NonIdealSource=off  SpecifyImpedance=off  Resistance=0  Inductance=0  ShortCircuitLevel=100e6  BaseVoltage=20e3  XRratio=7  BusType=PV  Pref=0  Qref=0  Prefabc=[10e3, 10e3, 10e3]  Qrefabc=[0, 0, 0]  Qmin=-inf  Qmax=inf
  fake_VSC_410 : powerlib/Electrical Sources/Three-Phase Source  Commented=on  InternalConnection=Yg  VoltagePhases=off  Voltage=(20000)*1  PhaseAngle=2.8249  Voltage_phases=[25e3 25e3 25e3]/sqrt(3)  PhaseAngles_phases=[0 -120 +120]  Frequency=50  NonIdealSource=off  SpecifyImpedance=off  Resistance=0  Inductance=0  ShortCircuitLevel=100e6  BaseVoltage=20e3  XRratio=7  BusType=PV  Pref=0  Qref=0  Prefabc=[10e3, 10e3, 10e3]  Qrefabc=[0, 0, 0]  Qmin=-inf  Qmax=inf
  fake_VSC_502 : powerlib/Electrical Sources/Three-Phase Source  Commented=on  InternalConnection=Yg  VoltagePhases=off  Voltage=(20000)*1  PhaseAngle=-12.7055  Voltage_phases=[25e3 25e3 25e3]/sqrt(3)  PhaseAngles_phases=[0 -120 +120]  Frequency=50  NonIdealSource=off  SpecifyImpedance=off  Resistance=0  Inductance=0  ShortCircuitLevel=100e6  BaseVoltage=20e3  XRratio=7  BusType=PV  Pref=0  Qref=0  Prefabc=[10e3, 10e3, 10e3]  Qrefabc=[0, 0, 0]  Qmin=-inf  Qmax=inf
  fake_VSC_504 : powerlib/Electrical Sources/Three-Phase Source  Commented=on  InternalConnection=Yg  VoltagePhases=off  Voltage=(20000)*1  PhaseAngle=-12.4459  Voltage_phases=[25e3 25e3 25e3]/sqrt(3)  PhaseAngles_phases=[0 -120 +120]  Frequency=50  NonIdealSource=off  SpecifyImpedance=off  Resistance=0  Inductance=0  ShortCircuitLevel=100e6  BaseVoltage=20e3  XRratio=7  BusType=PV  Pref=0  Qref=0  Prefabc=[10e3, 10e3, 10e3]  Qrefabc=[0, 0, 0]  Qmin=-inf  Qmax=inf
  fake_VSC_508 : powerlib/Electrical Sources/Three-Phase Source  Commented=on  InternalConnection=Yg  VoltagePhases=off  Voltage=(15000)*1  PhaseAngle=-14.7643  Voltage_phases=[25e3 25e3 25e3]/sqrt(3)  PhaseAngles_phases=[0 -120 +120]  Frequency=50  NonIdealSource=off  SpecifyImpedance=off  Resistance=0  Inductance=0  ShortCircuitLevel=100e6  BaseVoltage=20e3  XRratio=7  BusType=PV  Pref=0  Qref=0  Prefabc=[10e3, 10e3, 10e3]  Qrefabc=[0, 0, 0]  Qmin=-inf  Qmax=inf
  powergui : powerlib/powergui  Priority=1  SimulationMode=Phasor  SampleTime=50e-6  frequency=50  Iterations=50  frequencyindice=50  Pbase=100e6  ErrMax=0.0001  UnitsV=kV  UnitsW=MW  buscounter=0  FunctionMessages=off  echomessages=off  EnableUseOfTLC=off  CurrentSourceSwitches=off  DisableSnubberDevices=off  DisableRonSwitches=off  DisableVfSwitches=off  DisplayEquations=off  SolverType=Tustin  Interpol=off  ExternalGateDelay=off  methode=off  Ts=100  x0status=blocks  SPID=off  SwTol=0  HookPort=off  RestoreLinks=warning  ResistiveCurrentMeasurement=off  Frange=[0:2:500]  Ylog=off  Xlog=on  ShowGrid=off  save=off  variable=ZData  structure=0  ZoomFFT=off  StartTime=0.0  cycles=1  DisplayStyle=1  fundamental=60  FreqAxis=off  MaxFrequency=1000  frequencyindicesteady=1  RmsSteady=1  display=off
  u{102,208,212,215..216,308..309,312,314,403,405,410,502,504,508} (15 alike) : Constant  Value=0
  tag scope: P102=global, P208=global, P212=global, P215=global, P216=global, P308=global, P309=global, P312=global, P314=global, P403=global, P405=global, P410=global, P502=global, P504=global, P508=global, PSSmodel=global, Q102=global, Q208=global, Q212=global, Q215=global, Q216=global, Q308=global, Q309=global, Q312=global, Q314=global, Q403=global, Q405=global, Q410=global, Q502=global, Q504=global, Q508=global, w102=global, w208=global, w212=global, w215=global, w216=global, w308=global, w309=global, w312=global, w314=global, w403=global, w405=global, w410=global, w502=global, w504=global, w508=global
  wires:
  Demux/1 -> P 4-2/1
  Demux/2 -> P 4-2/2
  3-Phase Active & Reactive Power (Phasor Type)1/1 -> Demux/1
  Three-Phase V-I Measurement1/2 -> 3-Phase Active & Reactive Power (Phasor Type)1/2
  Three-Phase V-I Measurement1/1 -> 3-Phase Active & Reactive Power (Phasor Type)1/1
  Demux1/1 -> P 2-1/1
  Three-Phase V-I Measurement2/2 -> 3-Phase Active & Reactive Power (Phasor Type)2/2
  Three-Phase V-I Measurement2/1 -> 3-Phase Active & Reactive Power (Phasor Type)2/1
  3-Phase Active & Reactive Power (Phasor Type)2/1 -> Demux1/1
  Demux1/2 -> P 2-1/2
  Demux2/1 -> P 1-3/1
  3-Phase Active & Reactive Power (Phasor Type)3/1 -> Demux2/1
  Demux2/2 -> P 1-3/2
  Three-Phase V-I Measurement3/1 -> 3-Phase Active & Reactive Power (Phasor Type)3/1
  Three-Phase V-I Measurement3/2 -> 3-Phase Active & Reactive Power (Phasor Type)3/2
  Demux3/1 -> P 3-5/1
  3-Phase Active & Reactive Power (Phasor Type)4/1 -> Demux3/1
  Demux3/2 -> P 3-5/2
  Three-Phase V-I Measurement4/2 -> 3-Phase Active & Reactive Power (Phasor Type)4/2
  Three-Phase V-I Measurement4/1 -> 3-Phase Active & Reactive Power (Phasor Type)4/1
  PSS model/1 -> [PSSmodel]
  Voltage Measurement/1 -> Scope/1
  INV403/1 -> [P403]
  INV403/3 -> Mux15/2
  INV403/2 -> Mux15/1
  INV405/1 -> [P405]
  INV405/2 -> Mux16/1
  INV312/1 -> [P312]
  INV309/1 -> [P309]
  INV102/1 -> [P102]
  INV215/1 -> [P215]
  INV208/1 -> [P208]
  INV212/1 -> [P212]
  INV216/1 -> [P216]
  INV504/1 -> [P504]
  INV502/1 -> [P502]
  INV308/1 -> [P308]
  INV314/1 -> [P314]
  INV508/1 -> [P508]
  Mux15/1 -> [w403]
  Mux16/1 -> [w405]
  INV405/3 -> Mux16/2
  INV312/3 -> Mux17/2
  Mux17/1 -> [w312]
  INV312/2 -> Mux17/1
  INV314/3 -> Mux18/2
  Mux18/1 -> [w314]
  INV314/2 -> Mux18/1
  INV308/3 -> Mux19/2
  Mux19/1 -> [w308]
  INV308/2 -> Mux19/1
  INV508/3 -> Mux20/2
  Mux20/1 -> [w508]
  INV508/2 -> Mux20/1
  INV504/3 -> Mux21/2
  Mux21/1 -> [w504]
  INV504/2 -> Mux21/1
  INV502/3 -> Mux22/2
  Mux22/1 -> [w502]
  INV502/2 -> Mux22/1
  INV216/3 -> Mux23/2
  Mux23/1 -> [w216]
  INV216/2 -> Mux23/1
  INV410/3 -> Mux24/2
  Mux24/1 -> [w410]
  INV410/2 -> Mux24/1
  INV208/3 -> Mux25/2
  Mux25/1 -> [w208]
  INV208/2 -> Mux25/1
  INV212/3 -> Mux26/2
  Mux26/1 -> [w212]
  INV212/2 -> Mux26/1
  INV102/3 -> Mux27/2
  Mux27/1 -> [w102]
  INV102/2 -> Mux27/1
  INV309/3 -> Mux28/2
  Mux28/1 -> [w309]
  INV309/2 -> Mux28/1
  INV215/3 -> Mux29/2
  Mux29/1 -> [w215]
  INV215/2 -> Mux29/1
  INV403/4 -> Mux15/3
  INV216/4 -> Mux23/3
  u403/1 -> INV403/1
  u410/1 -> INV410/1
  u215/1 -> INV215/1
  u216/1 -> INV216/1
  u504/1 -> INV504/1
  u502/1 -> INV502/1
  u508/1 -> INV508/1
  u308/1 -> INV308/1
  u314/1 -> INV314/1
  u312/1 -> INV312/1
  u309/1 -> INV309/1
  u102/1 -> INV102/1
  u212/1 -> INV212/1
  u208/1 -> INV208/1
  u405/1 -> INV405/1
  INV212/4 -> Mux26/3
  INV410/1 -> [P410]
  INV405/4 -> Mux16/3
  INV410/4 -> Mux24/3
  INV215/4 -> Mux29/3
  INV504/4 -> Mux21/3
  INV502/4 -> Mux22/3
  INV508/4 -> Mux20/3
  INV308/4 -> Mux19/3
  INV314/4 -> Mux18/3
  INV312/4 -> Mux17/3
  INV309/4 -> Mux28/3
  INV102/4 -> Mux27/3
  INV208/4 -> Mux25/3
  [Pe401] -> Scope1/1
  Demux4/2 -> Scope4/2
  3-Phase Active & Reactive Power (Phasor Type)5/1 -> Demux4/1
  Demux4/1 -> Scope4/1
  Three-Phase V-I Measurement5/2 -> 3-Phase Active & Reactive Power (Phasor Type)5/2
  Three-Phase V-I Measurement5/1 -> 3-Phase Active & Reactive Power (Phasor Type)5/1
  INV504/5 -> [Q504]
  INV502/5 -> [Q502]
  INV216/5 -> [Q216]
  INV405/5 -> [Q405]
  INV403/5 -> [Q403]
  INV410/5 -> [Q410]
  INV215/5 -> [Q215]
  INV508/5 -> [Q508]
  INV308/5 -> [Q308]
  INV314/5 -> [Q314]
  INV312/5 -> [Q312]
  INV309/5 -> [Q309]
  INV102/5 -> [Q102]
  INV212/5 -> [Q212]
  INV208/5 -> [Q208]
  connections:
  L-38-1/LConn1 -- L-35-1/LConn1 -- L-35-2/LConn1 -- B406/RConn1 -- L-38-2/LConn1
  B406/RConn2 -- L-35-1/LConn2 -- L-35-2/LConn2 -- L-38-1/LConn2 -- L-38-2/LConn2
  L-35-1/LConn3 -- L-35-2/LConn3 -- B406/RConn3 -- L-38-1/LConn3 -- L-38-2/LConn3
  B407/RConn1 -- L-38-1/RConn1 -- L-38-2/RConn1
  B407/RConn2 -- L-38-1/RConn2 -- L-38-2/RConn2
  B407/RConn3 -- L-38-1/RConn3 -- L-38-2/RConn3
  B405/RConn1 -- L-35-2/RConn1 -- L-35-1/RConn1 -- T17/RConn1
  B405/RConn2 -- L-35-2/RConn2 -- L-35-1/RConn2 -- T17/RConn2
  B405/RConn3 -- L-35-2/RConn3 -- L-35-1/RConn3 -- T17/RConn3
  B407/LConn1 -- Load20/LConn1 -- L-39/LConn1 -- T16/RConn1
  B407/LConn2 -- Load20/LConn2 -- L-39/LConn2 -- T16/RConn2
  B407/LConn3 -- Load20/LConn3 -- L-39/LConn3 -- T16/RConn3
  T15/RConn1 -- B408/RConn1 -- L-39/RConn1 -- L-36-1/RConn1
  B408/RConn2 -- L-39/RConn2 -- L-36-1/RConn2 -- T15/RConn2
  B408/RConn3 -- L-39/RConn3 -- L-36-1/RConn3 -- T15/RConn3
  B405/LConn1 -- L-36-1/LConn1 -- T33/RConn1 -- Load18/LConn1 -- L-37-2/LConn1 -- L-37-3/LConn1 -- L-37-1/LConn1
  B405/LConn2 -- T33/RConn2 -- Load18/LConn2 -- L-37-2/LConn2 -- L-37-3/LConn2 -- L-36-1/LConn2 -- L-37-1/LConn2
  T33/RConn3 -- Load18/LConn3 -- L-37-2/LConn3 -- L-37-3/LConn3 -- L-36-1/LConn3 -- B405/LConn3 -- L-37-1/LConn3
  L-37-2/RConn1 -- L-37-1/RConn1 -- B409/RConn1 -- L-37-3/RConn1
  L-37-2/RConn2 -- L-37-1/RConn2 -- B409/RConn2 -- L-37-3/RConn2
  B409/RConn3 -- L-37-2/RConn3 -- L-37-3/RConn3 -- L-37-1/RConn3
  B409/LConn1 -- Load22/LConn1 -- Comp4-409/LConn1 -- L-41-2/LConn1 -- L-41-1/LConn1
  B409/LConn2 -- Comp4-409/LConn2 -- Load22/LConn2 -- L-41-2/LConn2 -- L-41-1/LConn2
  B409/LConn3 -- Comp4-409/LConn3 -- Load22/LConn3 -- L-41-2/LConn3 -- L-41-1/LConn3
  B408/LConn1 -- Load21/LConn1 -- L-40-2/LConn1 -- L-40-1/LConn1
  Load21/LConn2 -- L-40-2/LConn2 -- B408/LConn2 -- L-40-1/LConn2
  B408/LConn3 -- Load21/LConn3 -- L-40-2/LConn3 -- L-40-1/LConn3
  B411/RConn1 -- L-42/RConn1 -- L-41-2/RConn1 -- L-41-1/RConn1 -- T36/RConn1
  L-41-2/RConn2 -- L-41-1/RConn2 -- T36/RConn2 -- L-42/RConn2 -- B411/RConn2
  B411/RConn3 -- L-42/RConn3 -- T36/RConn3 -- L-41-2/RConn3 -- L-41-1/RConn3
  T14/RConn1 -- L-40-1/RConn1 -- L-40-2/RConn1 -- B410/RConn1
  B410/RConn2 -- L-40-2/RConn2 -- L-40-1/RConn2 -- T14/RConn2
  T14/RConn3 -- L-40-2/RConn3 -- L-40-1/RConn3 -- B410/RConn3
  T32/RConn1 -- L-44-1/LConn1 -- L-44-2/LConn1 -- L-43-1/LConn1 -- L-43-2/LConn1 -- L-43-3/LConn1 -- T35/RConn1 -- Voltage Measurement/LConn2 -- Load23/LConn1 -- L-42/LConn1 -- L-43-4/LConn1 -- B410/LConn1
  T32/RConn2 -- L-44-1/LConn2 -- L-44-2/LConn2 -- L-43-1/LConn2 -- L-43-2/LConn2 -- L-43-3/LConn2 -- L-43-4/LConn2 -- Load23/LConn2 -- Voltage Measurement/LConn1 -- L-42/LConn2 -- T35/RConn2 -- B410/LConn2
  L-44-1/LConn3 -- T32/RConn3 -- L-43-3/LConn3 -- T35/RConn3 -- L-42/LConn3 -- Load23/LConn3 -- L-43-4/LConn3 -- B410/LConn3 -- L-43-2/LConn3 -- L-43-1/LConn3 -- L-44-2/LConn3
  B413/RConn1 -- L-44-2/RConn1 -- L-44-1/RConn1
  B413/RConn2 -- L-44-2/RConn2 -- L-44-1/RConn2
  B413/RConn3 -- L-44-2/RConn3 -- L-44-1/RConn3
  B411/LConn1 -- Comp5-411/LConn1 -- Load24/LConn1 -- L-45-2/LConn1 -- L-45-1/LConn1
  B411/LConn2 -- Comp5-411/LConn2 -- Load24/LConn2 -- L-45-2/LConn2 -- L-45-1/LConn2
  B411/LConn3 -- Comp5-411/LConn3 -- Load24/LConn3 -- L-45-2/LConn3 -- L-45-1/LConn3
  B412/RConn1 -- L-45-2/RConn1 -- L-45-1/RConn1 -- L-43-4/RConn1 -- L-43-3/RConn1 -- L-43-1/RConn1 -- L-43-2/RConn1
  B412/RConn2 -- L-45-2/RConn2 -- L-45-1/RConn2 -- L-43-4/RConn2 -- L-43-3/RConn2 -- L-43-1/RConn2 -- L-43-2/RConn2
  L-43-3/RConn3 -- L-43-1/RConn3 -- L-43-2/RConn3 -- L-45-2/RConn3 -- L-45-1/RConn3 -- L-43-4/RConn3 -- B412/RConn3
  Load25/LConn1 -- B412/LConn1
  Load25/LConn2 -- B412/LConn2
  Load25/LConn3 -- B412/LConn3
  B404/LConn3 -- T17/LConn3
  B404/LConn2 -- T17/LConn2
  B404/LConn1 -- T17/LConn1
  Load Flow Bus2/LConn1 -- B404/RConn3 -- G404_GPS/LConn3
  B403_vi/RConn2 -- T16/LConn2
  B403_vi/RConn1 -- T16/LConn1
  B403_vi/RConn3 -- T16/LConn3
  20kV 2000MVA14/RConn3 -- 20kV 2000MVA1/RConn3 -- CPS403/LConn3 -- B403_vi/LConn3 -- Load Flow Bus15/LConn1
  B402/RConn2 -- T15/LConn2
  Load Flow Bus3/LConn1 -- B402/LConn1 -- CPS402/LConn1
  B402/RConn3 -- T15/LConn3
  B402/RConn1 -- T15/LConn1
  B401/RConn2 -- T14/LConn2
  B401/RConn3 -- T14/LConn3
  B401/RConn1 -- T14/LConn1
  G401_TPS/LConn1 -- B401/LConn1 -- Load Flow Bus4/LConn1
  G401_TPS/LConn2 -- B401/LConn2
  G401_TPS/LConn3 -- B401/LConn3
  B413/LConn1 -- T18-2/LConn1 -- T18-1/LConn1
  B413/LConn2 -- T18-2/LConn2 -- T18-1/LConn2
  B413/LConn3 -- T18-2/LConn3 -- T18-1/LConn3
  B414/RConn2 -- T18-2/RConn2 -- T18-1/RConn2
  B414/RConn1 -- T18-2/RConn1 -- T18-1/RConn1
  B414/RConn3 -- T18-2/RConn3 -- T18-1/RConn3
  B415/RConn1 -- L-46-2/RConn1 -- L-46-1/RConn1
  B415/RConn2 -- L-46-2/RConn2 -- L-46-1/RConn2
  B415/RConn3 -- L-46-2/RConn3 -- L-46-1/RConn3
  B414/LConn1 -- Comp6-414/LConn1 -- L-46-2/LConn1 -- L-46-1/LConn1
  Comp6-414/LConn2 -- B414/LConn2 -- L-46-1/LConn2 -- L-46-2/LConn2
  B414/LConn3 -- Comp6-414/LConn3 -- L-46-2/LConn3 -- L-46-1/LConn3
  L-6-1/RConn1 -- Three-Phase V-I Measurement1/LConn1 -- L-6-2/RConn1
  L-6-1/RConn2 -- L-6-2/RConn2 -- Three-Phase V-I Measurement1/LConn2
  L-6-1/RConn3 -- L-6-2/RConn3 -- Three-Phase V-I Measurement1/LConn3
  B416/LConn1 -- Comp8-416/LConn1 -- L-6-2/LConn1 -- L-6-1/LConn1
  B416/LConn2 -- Comp8-416/LConn2 -- L-6-2/LConn2 -- L-6-1/LConn2
  B416/LConn3 -- Comp8-416/LConn3 -- L-6-2/LConn3 -- L-6-1/LConn3
  L-7-1/RConn1 -- T37/RConn1 -- B206/RConn1 -- L-5-1/RConn1 -- L-5-2/RConn1 -- T2/RConn1 -- L-7-2/RConn1
  B206/RConn2 -- T37/RConn2 -- L-7-1/RConn2 -- L-7-2/RConn2 -- T2/RConn2 -- L-5-2/RConn2 -- L-5-1/RConn2
  T2/RConn3 -- L-7-1/RConn3 -- L-7-2/RConn3 -- T37/RConn3 -- L-5-2/RConn3 -- L-5-1/RConn3 -- B206/RConn3
  Load2/LConn1 -- L-5-1/LConn1 -- B205/LConn1 -- L-5-2/LConn1
  Load2/LConn2 -- L-5-1/LConn2 -- B205/LConn2 -- L-5-2/LConn2
  Load2/LConn3 -- L-5-1/LConn3 -- L-5-2/LConn3 -- B205/LConn3
  G201_BPS/LConn1 -- B201/RConn1
  B201/LConn1 -- T2/LConn1
  G201_BPS/LConn3 -- Load Flow Bus6/LConn1 -- B201/RConn3
  B201/LConn2 -- T2/LConn2
  B201/LConn3 -- T2/LConn3
  G201_BPS/LConn2 -- B201/RConn2
  B207/LConn1 -- L-11/LConn1 -- L-7-2/LConn1 -- L-7-1/LConn1
  B207/LConn2 -- L-11/LConn2 -- L-7-2/LConn2 -- L-7-1/LConn2
  B207/LConn3 -- L-11/LConn3 -- L-7-2/LConn3 -- L-7-1/LConn3
  B207/RConn1 -- L-10-2/RConn1 -- L-10-1/RConn1 -- Load4/LConn1
  B207/RConn2 -- L-10-2/RConn2 -- L-10-1/RConn2 -- Load4/LConn2
  B207/RConn3 -- L-10-2/RConn3 -- L-10-1/RConn3 -- Load4/LConn3
  T4/RConn1 -- T31/RConn1 -- L-10-1/LConn1 -- L-10-2/LConn1 -- B208/RConn1
  T4/RConn2 -- T31/RConn2 -- L-10-1/LConn2 -- L-10-2/LConn2 -- B208/RConn2
  T4/RConn3 -- T31/RConn3 -- L-10-1/LConn3 -- L-10-2/LConn3 -- B208/RConn3
  G203_VPS/LConn1 -- B203/RConn1
  B203/LConn1 -- T4/LConn1
  B203/LConn3 -- T4/LConn3
  G203_VPS/LConn2 -- B203/RConn2
  G203_VPS/LConn3 -- Load Flow Bus5/LConn1 -- B203/RConn3
  B203/LConn2 -- T4/LConn2
  L-12-3/LConn1 -- L-12-2/LConn1 -- L-12-1/LConn1 -- B211/RConn1
  L-12-3/LConn2 -- L-12-2/LConn2 -- L-12-1/LConn2 -- B211/RConn2
  L-12-3/LConn3 -- L-12-2/LConn3 -- B211/RConn3 -- L-12-1/LConn3
  Load5/LConn1 -- L-12-3/RConn1 -- L-12-2/RConn1 -- L-12-1/RConn1 -- B208/LConn1
  Load5/LConn2 -- L-12-3/RConn2 -- L-12-1/RConn2 -- B208/LConn2 -- L-12-2/RConn2
  Load5/LConn3 -- L-12-3/RConn3 -- L-12-2/RConn3 -- L-12-1/RConn3 -- B208/LConn3
  B211/LConn1 -- Load6/LConn1 -- L-16/RConn1 -- L-15-2/RConn1 -- L-15-1/RConn1
  L-16/RConn2 -- Load6/LConn2 -- L-15-2/RConn2 -- L-15-1/RConn2 -- B211/LConn2
  B211/LConn3 -- Load6/LConn3 -- L-16/RConn3 -- L-15-2/RConn3 -- L-15-1/RConn3
  B206/LConn1 -- L-9-1/RConn1 -- L-9-2/RConn1 -- Load3/LConn1 -- L-8-2/RConn1 -- L-8-1/RConn1
  L-9-1/RConn2 -- Load3/LConn2 -- L-8-2/RConn2 -- L-8-1/RConn2 -- B206/LConn2 -- L-9-2/RConn2
  B206/LConn3 -- L-9-1/RConn3 -- L-9-2/RConn3 -- Load3/LConn3 -- L-8-2/RConn3 -- L-8-1/RConn3
  L-15-2/LConn1 -- L-15-1/LConn1 -- T38/RConn1 -- L-8-1/LConn1 -- L-13/LConn1 -- B212/RConn1 -- L-8-2/LConn1
  B212/RConn2 -- L-13/LConn2 -- L-8-2/LConn2 -- T38/RConn2 -- L-15-2/LConn2 -- L-15-1/LConn2 -- L-8-1/LConn2
  L-15-2/LConn3 -- L-15-1/LConn3 -- T38/RConn3 -- L-8-2/LConn3 -- L-8-1/LConn3 -- L-13/LConn3 -- B212/RConn3
  T3/RConn3 -- L-11/RConn3 -- B209/RConn3
  T3/RConn2 -- L-11/RConn2 -- B209/RConn2
  T3/RConn1 -- L-11/RConn1 -- B209/RConn1
  B202/LConn2 -- T3/LConn2
  G202_EPS/LConn3 -- B202/RConn3
  B202/LConn3 -- T3/LConn3
  G202_EPS/LConn1 -- Load Flow Bus7/LConn1 -- B202/RConn1
  B202/LConn1 -- T3/LConn1
  G202_EPS/LConn2 -- B202/RConn2
  T6/LConn1 -- L-13/RConn1 -- B209/LConn1
  T6/LConn2 -- L-13/RConn2 -- B209/LConn2
  T6/LConn3 -- L-13/RConn3 -- B209/LConn3
  B210/RConn1 -- T6/RConn1
  B210/RConn2 -- T6/RConn2
  B210/RConn3 -- T6/RConn3
  B213/RConn1 -- L-14-1/LConn1 -- L-14-2/LConn1
  B213/RConn2 -- L-14-1/LConn2 -- L-14-2/LConn2
  B213/RConn3 -- L-14-1/LConn3 -- L-14-2/LConn3
  B210/LConn1 -- L-14-2/RConn1 -- L-14-1/RConn1
  B210/LConn2 -- L-14-2/RConn2 -- L-14-1/RConn2
  B210/LConn3 -- L-14-2/RConn3 -- L-14-1/RConn3
  L-17/RConn1 -- T28/RConn1 -- Comp2-212/LConn1 -- Load7/LConn1 -- B212/LConn1
  B212/LConn2 -- Load7/LConn2 -- T28/RConn2 -- Comp2-212/LConn2 -- L-17/RConn2
  B212/LConn3 -- Load7/LConn3 -- T28/RConn3 -- Comp2-212/LConn3 -- L-17/RConn3
  B214/RConn2 -- L-16/LConn2 -- T7/RConn2
  B214/RConn1 -- L-16/LConn1 -- T7/RConn1
  B214/RConn3 -- L-16/LConn3 -- T7/RConn3
  T7/LConn1 -- B213/LConn1
  T7/LConn2 -- B213/LConn2
  T7/LConn3 -- B213/LConn3
  L-18/LConn2 -- T29/RConn2 -- L-20-1/LConn2 -- L-20-2/LConn2 -- B216/RConn2
  L-18/LConn1 -- T29/RConn1 -- L-20-1/LConn1 -- L-20-2/LConn1 -- B216/RConn1
  L-18/LConn3 -- B216/RConn3 -- T29/RConn3 -- L-20-1/LConn3 -- L-20-2/LConn3
  B214/LConn3 -- L-19/RConn3 -- L-18/RConn3
  B214/LConn1 -- L-19/RConn1 -- L-18/RConn1
  B214/LConn2 -- L-19/RConn2 -- L-18/RConn2
  L-22/LConn1 -- L-19/LConn1 -- L-17/LConn1 -- L-21-2/LConn1 -- L-21-1/LConn1 -- B217/RConn1
  L-22/LConn2 -- L-19/LConn2 -- L-17/LConn2 -- L-21-1/LConn2 -- L-21-2/LConn2 -- B217/RConn2
  L-22/LConn3 -- L-19/LConn3 -- L-17/LConn3 -- L-21-1/LConn3 -- L-21-2/LConn3 -- B217/RConn3
  L-22/RConn1 -- Comp3-216/LConn1 -- Load9/LConn1 -- B216/LConn1
  L-22/RConn2 -- Comp3-216/LConn2 -- Load9/LConn2 -- B216/LConn2
  L-22/RConn3 -- Comp3-216/LConn3 -- Load9/LConn3 -- B216/LConn3
  B215/RConn1 -- L-9-2/LConn1 -- L-9-1/LConn1
  B215/RConn2 -- L-9-2/LConn2 -- L-9-1/LConn2
  B215/RConn3 -- L-9-2/LConn3 -- L-9-1/LConn3
  T5/RConn1 -- Load8/LConn1 -- T30/RConn1 -- L-21-1/RConn1 -- L-20-2/RConn1 -- L-20-1/RConn1 -- L-21-2/RConn1 -- B215/LConn1
  T5/RConn2 -- Load8/LConn2 -- L-21-1/RConn2 -- T30/RConn2 -- L-20-2/RConn2 -- L-20-1/RConn2 -- L-21-2/RConn2 -- B215/LConn2
  T5/RConn3 -- Load8/LConn3 -- L-21-1/RConn3 -- T30/RConn3 -- L-20-2/RConn3 -- L-20-1/RConn3 -- L-21-2/RConn3 -- B215/LConn3
  L-2-1/RConn1 -- L-1-1/RConn1 -- L-1-2/RConn1 -- L-2-2/RConn1 -- Three-Phase V-I Measurement2/LConn1
  L-2-2/RConn3 -- Three-Phase V-I Measurement2/LConn3 -- L-1-1/RConn3 -- L-1-2/RConn3 -- L-2-1/RConn3
  L-1-1/LConn1 -- B217/LConn1 -- Load10/LConn1 -- L-2-2/LConn1 -- L-2-1/LConn1 -- L-1-2/LConn1
  B217/LConn2 -- Load10/LConn2 -- L-2-2/LConn2 -- L-2-1/LConn2 -- L-1-2/LConn2 -- L-1-1/LConn2
  L-1-1/LConn3 -- Load10/LConn3 -- L-2-2/LConn3 -- L-2-1/LConn3 -- L-1-2/LConn3 -- B217/LConn3
  L-3-1/RConn1 -- L-4/RConn1 -- L-3-2/RConn1 -- Three-Phase V-I Measurement3/LConn1
  L-3-1/RConn2 -- L-4/RConn2 -- L-3-2/RConn2 -- Three-Phase V-I Measurement3/LConn2
  L-3-1/RConn3 -- L-4/RConn3 -- L-3-2/RConn3 -- Three-Phase V-I Measurement3/LConn3
  B102/LConn1 -- L-3-1/LConn1 -- T1/RConn1 -- Load1/LConn1 -- L-4/LConn1 -- L-3-2/LConn1
  B102/LConn2 -- L-3-1/LConn2 -- T1/RConn2 -- Load1/LConn2 -- L-4/LConn2 -- L-3-2/LConn2
  B102/LConn3 -- L-3-1/LConn3 -- T1/RConn3 -- Load1/LConn3 -- L-4/LConn3 -- L-3-2/LConn3
  B101/LConn1 -- T1/LConn1
  Load Flow Bus9/LConn1 -- Three-Phase V-I Measurement5/RConn3 -- B101/RConn3
  B101/LConn3 -- T1/LConn3
  B101/LConn2 -- T1/LConn2
  L-30-2/LConn2 -- B309/LConn2 -- Load14/LConn2 -- L-30-1/LConn2
  L-30-2/LConn3 -- B309/LConn3 -- Load14/LConn3 -- L-30-1/LConn3
  T11/LConn1 -- T12/LConn1 -- B305/RConn1 -- L-24-1/LConn1 -- L-24-2/LConn1 -- L-25/LConn1
  T11/LConn2 -- T12/LConn2 -- B305/RConn2 -- L-24-1/LConn2 -- L-24-2/LConn2 -- L-25/LConn2
  T11/LConn3 -- T12/LConn3 -- B305/RConn3 -- L-24-1/LConn3 -- L-24-2/LConn3 -- L-25/LConn3
  L-24-2/RConn1 -- L-24-1/RConn1 -- L-23/RConn1 -- B303/RConn1
  L-24-2/RConn2 -- L-24-1/RConn2 -- L-23/RConn2 -- B303/RConn2
  L-24-2/RConn3 -- L-24-1/RConn3 -- L-23/RConn3 -- B303/RConn3
  B307/RConn1 -- L-28/LConn1 -- T39/RConn1 -- L-27-2/LConn1 -- L-27-1/LConn1
  B307/RConn2 -- L-28/LConn2 -- T39/RConn2 -- L-27-2/LConn2 -- L-27-1/LConn2
  B307/RConn3 -- L-28/LConn3 -- T39/RConn3 -- L-27-2/LConn3 -- L-27-1/LConn3
  B305/LConn1 -- L-26/RConn1 -- L-27-2/RConn1 -- L-27-1/RConn1
  B305/LConn2 -- L-26/RConn2 -- L-27-2/RConn2 -- L-27-1/RConn2
  B305/LConn3 -- L-26/RConn3 -- L-27-2/RConn3 -- L-27-1/RConn3
  L-25/RConn1 -- B304/LConn1
  L-25/RConn2 -- B304/LConn2
  L-25/RConn3 -- B304/LConn3
  G301_LPS/LConn2 -- B301/LConn2
  G301_LPS/LConn1 -- B301/LConn1
  G301_LPS/LConn3 -- Load Flow Bus10/LConn1 -- B301/LConn3
  T8/LConn1 -- B301/RConn1
  T8/LConn3 -- B301/RConn3
